simulink library "allblocks_alteradspbuilder2"  (Simulink 7.6)
(part 2 of 4)

  GND : S-Function  LoadFcn=alt_dspbuilder_load_block(gcb, 'BlockFactory', 'com.altera.dspbuilder.blockset.iobus.GND');  FunctionName=sGeneric  Parameters=SpecifyClock  EnableBusSupport=off  mask(GND AlteraBlockset){SpecifyClock=off, clock=}
      mask prompts: SpecifyClock "Specify Clock"
      mask help: A single bit which outputs a constant 0 value.
      mask init:
      | alt_dspbuilder_init('BlockFactory', 'com.altera.dspbuilder.blockset.iobus.GND', { get_param(gcb, 'SpecifyClock') clock });
      settings: CopyFcn=alt_dspbuilder_add_block(gcb, 'BlockFactory', 'com.altera.dspbuilder.blockset.iobus.GND');  DeleteFcn=com.altera.dspbuilder.simulation.Mask.delete(gcb);  UndoDeleteFcn=alt_dspbuilder_add_block(gcb, 'BlockFactory', 'com.altera.dspbuilder.blockset.iobus.GND');  PostSaveFcn=alt_dspbuilder_block_saved(gcb);  NameChangeFcn=alt_dspbuilder_block_renamed(gcb);
      mask Help: helpview(char(com.altera.dspbuilder.simulation.Cache.getBlockTemplate('BlockFactory', 'com.altera.dspbuilder.blockset.iobus.GND').getHelpFile))
      mask CallbackString: alt_dspbuilder_update_gui('BlockFactory', 'com.altera.dspbuilder.blockset.iobus.GND', 'SpecifyClock', 0);|
      mask Display:
      | plot([1 0 0 1], [1 1 0 0])
      | disp('0');
  Gain : S-Function  LoadFcn=alt_dspbuilder_load_block(gcb, 'BlockFactory', 'com.altera.dspbuilder.blockset.arithmetic.Gain');  FunctionName=sGeneric  Parameters=vgain BusType bwl bwr pipeline pipeline_display allowFloatingPointOverride logOutputs logFile MaskValue use_ena use_aclr lpm  EnableBusSupport=off  mask(Gain AlteraBlockset){vgain=2, BusType=Signed Integer, bwl=8, bwr=0, pipeline=1, pipeline_display=1, allowFloatingPointOverride=on, logOutputs=off, logFile=D:\\allblocks%5Falteradspbuilder2_Gain.fixedpointlog, MaskValue=1, use_ena=off, use_aclr=off, lpm=off}
      mask prompts: vgain "Gain Value"; BusType "Map Gain Value to Bus Type"; bwl "[Gain Value Number Of Bits].[]"; bwr "[].[Gain Value Number Of Bits]"; pipeline "Number Of Pipeline Stages"; pipeline_display "Number Of Pipeline Stages (Calculated)"; allowFloatingPointOverride "Allow Floating Point Override For This Block"; MaskValue "Clock Phase Selection"; use_ena "Use Enable Port (ena)"; use_aclr "Use Asynchronous Clear Port (aclr)"; lpm "Use LPM"
      mask help: Multiplies an input by a specified scalar gain factor.
      mask init:
      | alt_dspbuilder_init('BlockFactory', 'com.altera.dspbuilder.blockset.arithmetic.Gain', { vgain get_param(gcb, 'BusType') bwl bwr pipeline pipeline_display allowFloatingPointOverride logOutputs logFile MaskValue use_ena use_aclr lpm });
      settings: CopyFcn=alt_dspbuilder_add_block(gcb, 'BlockFactory', 'com.altera.dspbuilder.blockset.arithmetic.Gain');  DeleteFcn=com.altera.dspbuilder.simulation.Mask.delete(gcb);  UndoDeleteFcn=alt_dspbuilder_add_block(gcb, 'BlockFactory', 'com.altera.dspbuilder.blockset.arithmetic.Gain');  PostSaveFcn=alt_dspbuilder_block_saved(gcb);  NameChangeFcn=alt_dspbuilder_block_renamed(gcb);
      mask Help: helpview(char(com.altera.dspbuilder.simulation.Cache.getBlockTemplate('BlockFactory', 'com.altera.dspbuilder.blockset.arithmetic.Gain').getHelpFile))
      mask StyleString: edit,popup(Signed Integer|Unsigned Integer|Signed Fractional|Unsigned Fractional),edit,edit,edit,edit,checkbox,checkbox,edit,edit,checkbox,checkbox,checkbox
      mask CallbackString: |alt_dspbuilder_update_gui('BlockFactory', 'com.altera.dspbuilder.blockset.arithmetic.Gain', 'BusType', 1);|||||||||||
      mask TabNameString: Main,Main,Main,Main,Main,Main,Main,Main,Main,Optional Ports and Settings,Optional Ports and Settings,Optional Ports and Settings,Optional Ports and Settings
      mask Display:
      | port_label('input', 1, 'd');
      | port_label('output', 1, 'r');
      | plot([0 0 0 1 0], [0 1 0 0.5 1])
      | disp(2);
  Global Reset : S-Function  LoadFcn=alt_dspbuilder_load_block(gcb, 'BlockFactory', 'com.altera.dspbuilder.blockset.iobus.GlobalReset');  FunctionName=sGeneric  Parameters=SpecifyClock  EnableBusSupport=off  mask(GlobalReset AlteraBlockset){SpecifyClock=off, clock=}
      mask prompts: SpecifyClock "Specify Clock"
      mask help: Provides a single bit reset signal. All signals driven by the block are connected to the global reset for that clock domain. In simulation, this block outputs a constant 0.
      mask init:
      | alt_dspbuilder_init('BlockFactory', 'com.altera.dspbuilder.blockset.iobus.GlobalReset', { get_param(gcb, 'SpecifyClock') get_param(gcb, 'clock') });
      settings: CopyFcn=alt_dspbuilder_add_block(gcb, 'BlockFactory', 'com.altera.dspbuilder.blockset.iobus.GlobalReset');  DeleteFcn=com.altera.dspbuilder.simulation.Mask.delete(gcb);  UndoDeleteFcn=alt_dspbuilder_add_block(gcb, 'BlockFactory', 'com.altera.dspbuilder.blockset.iobus.GlobalReset');  PostSaveFcn=alt_dspbuilder_block_saved(gcb);  NameChangeFcn=alt_dspbuilder_block_renamed(gcb);
      mask Help: helpview(char(com.altera.dspbuilder.simulation.Cache.getBlockTemplate('BlockFactory', 'com.altera.dspbuilder.blockset.iobus.GlobalReset').getHelpFile))
      mask CallbackString: alt_dspbuilder_update_gui('BlockFactory', 'com.altera.dspbuilder.blockset.iobus.GlobalReset', 'SpecifyClock', 0);|alt_dspbuilder_update_gui('BlockFactory', 'com.altera.dspbuilder.blockset.iobus.GlobalReset', 'clock', 1);
      mask Display:
      | plot([1 0 0 1], [1 1 0 0])
      | disp('SCLR');
  HDL Entity : S-Function  LoadFcn=alt_dspbuilder_load_block(gcb, 'BlockFactory', 'com.altera.dspbuilder.blockset.altlab.HDLEntity');  FunctionName=sNoOp  Parameters=HDLFile clockname resetname useSubsystemPortName  EnableBusSupport=off  mask(HDL Entity AlteraBlockset){HDLFile=, clockname=, resetname=, useSubsystemPortName=off}
      mask prompts: HDLFile "HDL File Name"; clockname "Clock Name"; resetname "Reset Name"; useSubsystemPortName "HDL takes port names from Subsystem Inport/Outports"
      mask help:
      | This block is added to a black box simulation subsystem to specify the name of the HDL file that is substituted for the subsystem and
      | the names of the clock and reset ports for the subsystem. A HDL Entity block is usually automatically created by the Subsystem Builder Block.
      mask init:
      | alt_dspbuilder_init('BlockFactory', 'com.altera.dspbuilder.blockset.altlab.HDLEntity', { HDLFile clockname resetname useSubsystemPortName });
      settings: CopyFcn=alt_dspbuilder_add_block(gcb, 'BlockFactory', 'com.altera.dspbuilder.blockset.altlab.HDLEntity');  DeleteFcn=com.altera.dspbuilder.simulation.Mask.delete(gcb);  UndoDeleteFcn=alt_dspbuilder_add_block(gcb, 'BlockFactory', 'com.altera.dspbuilder.blockset.altlab.HDLEntity');  PostSaveFcn=alt_dspbuilder_block_saved(gcb);  NameChangeFcn=alt_dspbuilder_block_renamed(gcb);
      mask Help: helpview(char(com.altera.dspbuilder.simulation.Cache.getBlockTemplate('BlockFactory', 'com.altera.dspbuilder.blockset.altlab.HDLEntity').getHelpFile))
      mask Display: disp('');
  HDL Input : S-Function  LoadFcn=alt_dspbuilder_load_block(gcb, 'BlockFactory', 'com.altera.dspbuilder.blockset.altlab.HDLInput');  FunctionName=sInOut  Parameters=BusType bwl bwr externalType  EnableBusSupport=off  mask(HDL Input AlteraBlockset){BusType=Signed Integer, bwl=8, bwr=0, externalType=Inferred}
      mask prompts: BusType "Bus Type"; bwl "[number of bits].[]"; bwr "[].[number of bits]"; externalType "External Type"
      mask help:
      | This block should be connected directly to an output node in a subsystem. It is intended to be used with the Subsystem Builder and HDL Entity blocks for black box simulation.
      |
      | The type and bit width must match the type and bit width on the corresponding input port in the HDL file specified in the HDL Entity block. HDL Input blocks are automatically created by the Subsystem Builder block.
      mask init:
      | alt_dspbuilder_init('BlockFactory', 'com.altera.dspbuilder.blockset.altlab.HDLInput', { get_param(gcb, 'BusType') bwl bwr externalType });
      settings: CopyFcn=alt_dspbuilder_add_block(gcb, 'BlockFactory', 'com.altera.dspbuilder.blockset.altlab.HDLInput');  DeleteFcn=com.altera.dspbuilder.simulation.Mask.delete(gcb);  UndoDeleteFcn=alt_dspbuilder_add_block(gcb, 'BlockFactory', 'com.altera.dspbuilder.blockset.altlab.HDLInput');  PostSaveFcn=alt_dspbuilder_block_saved(gcb);  NameChangeFcn=alt_dspbuilder_block_renamed(gcb);
      mask Help: helpview(char(com.altera.dspbuilder.simulation.Cache.getBlockTemplate('BlockFactory', 'com.altera.dspbuilder.blockset.altlab.HDLInput').getHelpFile))
      mask StyleString: popup(Signed Integer|Unsigned Integer|Signed Fractional|Unsigned Fractional|Single Bit),edit,edit,popup(Inferred|Simulink Fixed Point Type|Double)
      mask CallbackString: alt_dspbuilder_update_gui('BlockFactory', 'com.altera.dspbuilder.blockset.altlab.HDLInput', 'BusType', 0);|||
      mask Display:
      | plot([0.17 0 0.83 1 0.83 0 0.17], [0.5 0 0 0.5 1 1 0.5])
      | plot([0.07 0.23 0.07 0.77 0.93  0.77], [0 0.5 1 1 0.5 0])
      | disp('i7:0')
  HDL Output : S-Function  LoadFcn=alt_dspbuilder_load_block(gcb, 'BlockFactory', 'com.altera.dspbuilder.blockset.altlab.HDLOutput');  FunctionName=sInOut  Parameters=BusType bwl bwr externalType  EnableBusSupport=off  mask(HDL Output AlteraBlockset){BusType=Signed Integer, bwl=8, bwr=0, externalType=Inferred}
      mask prompts: BusType "Bus Type"; bwl "[number of bits].[]"; bwr "[].[number of bits]"; externalType "External Type"
      mask help:
      | This block should be connected directly to an input node in a subsystem. It is intended to be used with the Subsystem Builder and HDL Entity blocks for black box simulation.
      |
      | The type and bit width must match the type and bit width on the corresponding output port in the HDL file specified in the HDL Entity block. HDL Output blocks are automatically created by the Subsystem Builder block.
      mask init:
      | alt_dspbuilder_init('BlockFactory', 'com.altera.dspbuilder.blockset.altlab.HDLOutput', { get_param(gcb, 'BusType') bwl bwr externalType });
      settings: CopyFcn=alt_dspbuilder_add_block(gcb, 'BlockFactory', 'com.altera.dspbuilder.blockset.altlab.HDLOutput');  DeleteFcn=com.altera.dspbuilder.simulation.Mask.delete(gcb);  UndoDeleteFcn=alt_dspbuilder_add_block(gcb, 'BlockFactory', 'com.altera.dspbuilder.blockset.altlab.HDLOutput');  PostSaveFcn=alt_dspbuilder_block_saved(gcb);  NameChangeFcn=alt_dspbuilder_block_renamed(gcb);
      mask Help: helpview(char(com.altera.dspbuilder.simulation.Cache.getBlockTemplate('BlockFactory', 'com.altera.dspbuilder.blockset.altlab.HDLOutput').getHelpFile))
      mask StyleString: popup(Signed Integer|Unsigned Integer|Signed Fractional|Unsigned Fractional|Single Bit),edit,edit,popup(Inferred|Simulink Fixed Point Type|Double)
      mask CallbackString: alt_dspbuilder_update_gui('BlockFactory', 'com.altera.dspbuilder.blockset.altlab.HDLOutput', 'BusType', 0);|||
      mask Display:
      | plot([0 0.17 1 0.83 1 0.17 0], [0.5 0 0 0.5 1 1 0.5])
      | plot([0.23 0.07 0.23 0.93 0.77 0.93], [0 0.5 1 1 0.5 0])
      | disp('o7:0')
  HDLImport : S-Function  LoadFcn=alt_dspbuilder_load_block(gcb, 'BlockFactory', 'com.altera.dspbuilder.blockset.altlab.HDLImport');  InitFcn=alt_dspbuilder_internal_init_blackbox_flow;  FunctionName=sGeneric  Parameters=entityName inNames inBwls inBwrs inTypes inDelayed outNames outBwls outBwrs outTypes resetNames resetTypes resetLengths xmlmapfile vofile src_file qpf_file TopLevelName UseQPF n_input_port n_output_port array_clocks use_systemC_model is_megacore use_dynamic_feedthrough_data use_alphabetical_port_ordering allowFloatingPointOverride  EnableBusSupport=off  mask(HDLImport AlteraBlockset){entityName=, inNames=, inBwls=, inBwrs=, inTypes=, inDelayed=, outNames=, outBwls=, outBwrs=, outTypes=, resetNames=, resetTypes=, resetLengths=, xmlmapfile=SimgenCMap.xml, vofile=test_core.vo, src_file=, qpf_file=, TopLevelName=, UseQPF=false, n_input_port=0, n_output_port=0, array_clocks=, use_systemC_model=off, is_megacore=off, use_dynamic_feedthrough_data=off, use_alphabetical_port_ordering=, allowFloatingPointOverride=off}
      mask prompts: entityName "Entity Name"; inNames "Input port names"; inBwls "Input Bitwidth lefts"; inBwrs "Input Bitwidth rights"; inTypes "Input Types"; inDelayed "Input Delayed Flags"; outNames "Output port names"; outBwls "Output Bitwidth lefts"; outBwrs "Output Bitwidth rights"; outTypes "Output Types"; resetNames "array_clocks"; resetTypes "array_clocks"; resetLengths "array_clocks"; use_systemC_model "Use SystemC bit-accurate model"
      mask help: Used to import supported VHDL or Verilog HDL components into DSP Builder, generating hardware and simulation models as required. You can either specify the HDL files directly, or select a Quartus II project file (.qpf) that defines the required HDL files. The HDL Import dialog box must be closed before simulation can start.
      mask init:
      | alt_dspbuilder_init('BlockFactory', 'com.altera.dspbuilder.blockset.altlab.HDLImport', { entityName inNames inBwls inBwrs inTypes inDelayed outNames outBwls outBwrs outTypes resetNames resetTypes resetLengths xmlmapfile vofile src_file qpf_file TopLevelName UseQPF n_input_port n_output_port array_clocks use_systemC_model is_megacore use_dynamic_feedthrough_data use_alphabetical_port_ordering allowFloatingPointOverride });
      settings: CopyFcn=alt_dspbuilder_add_block(gcb, 'BlockFactory', 'com.altera.dspbuilder.blockset.altlab.HDLImport');  DeleteFcn=com.altera.dspbuilder.simulation.Mask.delete(gcb);  UndoDeleteFcn=alt_dspbuilder_add_block(gcb, 'BlockFactory', 'com.altera.dspbuilder.blockset.altlab.HDLImport');  PostSaveFcn=alt_dspbuilder_block_saved(gcb);  NameChangeFcn=alt_dspbuilder_block_renamed(gcb);
      settings: OpenFcn=|
      | com.altera.dspbuilder.simulation.Mask.simpleInit('BlockFactory', 'com.altera.dspbuilder.blockset.altlab.HDLImport', bdroot(gcb), gcb);
      | alt_dspbuilder_internal_HDLimportlaunch(gcb, 0)
      mask Help: helpview(char(com.altera.dspbuilder.simulation.Cache.getBlockTemplate('BlockFactory', 'com.altera.dspbuilder.blockset.altlab.HDLImport').getHelpFile))
      mask Display: disp('HDL')
  HIL : S-Function  LoadFcn=alt_dspbuilder_load_block(gcb, 'BlockFactory', 'com.altera.dspbuilder.blockset.altlab.HardwareInTheLoop');  FunctionName=sGeneric  Parameters=entityName inNames inBwls inBwrs inTypes inDelayed outNames outBwls outBwrs outTypes resetNames resetTypes resetLengths InputCount InputNames InputWidth InputRepresentation InputExport InputFPP OutputCount OutputNames OutputWidth OutputRepresentation OutputExport OutputFPP JtagCable JtagDevice BurstMode BurstLength FrameMode SOP OutValid QuartusProject HilNewConfig ClockPinLocation ClockPinSource HilDeviceOnBoard DR_length dspbuilder_reset SLD_NODE_INFO AssertSclrBeforeSimulation SampleTime dspb_ver ResetLevel JtagCableName JtagDeviceName ResetNames ClockNames  EnableBusSupport=off  mask(HardwareInTheLoop AlteraBlockset){entityName=, inNames=, inBwls=, inBwrs=, inTypes=, inDelayed=, outNames=, outBwls=, outBwrs=, outTypes=, resetNames=, resetTypes=, resetLengths=, InputCount=0, InputNames=, InputWidth=0, InputRepresentation=b, InputExport=0, InputFPP=0, OutputCount=0, OutputNames=, OutputWidth=0, OutputRepresentation=0, OutputExport=0, OutputFPP=0, JtagCable=1, JtagDevice=1, BurstMode=off, BurstLength=0, FrameMode=off, SOP=0, OutValid=0, QuartusProject=0, HilNewConfig=0, ClockPinLocation=0, ClockPinSource=0, HilDeviceOnBoard=0, DR_length=0, dspbuilder_reset=1, SLD_NODE_INFO=0, AssertSclrBeforeSimulation=0, SampleTime=0, dspb_ver=0, ResetLevel=Active_High, JtagCableName=a, JtagDeviceName=b, ResetNames=, ClockNames=}
      mask prompts: entityName "Entity Name"; inNames "Input port names"; inBwls "Input Bitwidth lefts"; inBwrs "Input Bitwidth rights"; inTypes "Input Types"; inDelayed "Input Delayed Flags"; outNames "Output port names"; outBwls "Output Bitwidth lefts"; outBwrs "Output Bitwidth rights"; outTypes "Output Types"; resetNames "array_clocks"; resetTypes "array_clocks"; resetLengths "array_clocks"; InputCount "Input Count"; InputNames "Input Names"; InputWidth "Input Width"; InputRepresentation "Input Representation"; InputExport "Input Export"; InputFPP "Input FPP"; OutputCount "Output Count"; OutputNames "Output Names"; OutputWidth "Output Width"; OutputRepresentation "Output Representation"; OutputExport "Output Export"; OutputFPP "Output FPP"; JtagCable "JTAG Cable"; JtagDevice "JTAG Device"; BurstMode "Burst Mode"; BurstLength "Burst Length"; FrameMode "Frame Mode"; OutValid "Out Valid"; QuartusProject "Quartus Project"; HilNewConfig "HIL New Config"; ClockPinLocation "Clock Pin Location"; ClockPinSource "Clock Pin Source"; HilDeviceOnBoard "Hil Device On Board"; DR_length "DR Length"; dspbuilder_reset "DSP Builder Reset"; SLD_NODE_INFO "SLD NODE INFO"; AssertSclrBeforeSimulation "Assert Sclr Before Simulation"; SampleTime "Sample Time"; dspb_ver "DSP Builder Version"; ResetLevel "Reset Level"; JtagCableName "JTAG Cable Name"; JtagDeviceName "JTAG Device Name"; ResetNames "Reset Names"; ClockNames "Clock Names"
      mask help: The HIL (Hardware In the Loop) block allows you to use an FPGA as a simulation device inside a Simulink design. This configuration improves the simulation time, and also allows access to real hardware within a simulation.
      mask init:
      | alt_dspbuilder_init_hil('BlockFactory', 'com.altera.dspbuilder.blockset.altlab.HardwareInTheLoop', { entityName inNames inBwls inBwrs inTypes inDelayed outNames outBwls outBwrs outTypes resetNames resetTypes resetLengths InputCount InputNames InputWidth InputRepresentation InputExport InputFPP OutputCount OutputNames OutputWidth OutputRepresentation OutputExport OutputFPP JtagCable JtagDevice BurstMode BurstLength FrameMode SOP OutValid QuartusProject HilNewConfig ClockPinLocation ClockPinSource HilDeviceOnBoard DR_length dspbuilder_reset SLD_NODE_INFO AssertSclrBeforeSimulation SampleTime dspb_ver ResetLevel JtagCableName JtagDeviceName ResetNames ClockNames });
      settings: CopyFcn=alt_dspbuilder_add_block(gcb, 'BlockFactory', 'com.altera.dspbuilder.blockset.altlab.HardwareInTheLoop');  DeleteFcn=com.altera.dspbuilder.simulation.Mask.delete(gcb);  UndoDeleteFcn=alt_dspbuilder_add_block(gcb, 'BlockFactory', 'com.altera.dspbuilder.blockset.altlab.HardwareInTheLoop');  PostSaveFcn=alt_dspbuilder_block_saved(gcb);  NameChangeFcn=alt_dspbuilder_block_renamed(gcb);
      settings: OpenFcn=|
      | com.altera.dspbuilder.simulation.Mask.simpleInit('BlockFactory', 'com.altera.dspbuilder.blockset.altlab.HardwareInTheLoop', bdroot(gcb), gcb);
      | alt_dspbuilder_HilConfig('BLOCKNAME', gcb)
      mask Help: helpview(char(com.altera.dspbuilder.simulation.Cache.getBlockTemplate('BlockFactory', 'com.altera.dspbuilder.blockset.altlab.HardwareInTheLoop').getHelpFile))
      mask Display:
      | plot([-20],[0]);
      | plot([23],[26]);
      | plot([0 4 3 5 3 1 2 0],[0 3 3 6 6 3 3 0]);
      | plot([0 4 3 5 3 1 2 0],[20 23 23 26 26 23 23 20]);
      | disp(entityName);
  If Statement : S-Function  LoadFcn=alt_dspbuilder_load_block(gcb, 'BlockFactory', 'com.altera.dspbuilder.blockset.gatecontrol.IfStatement');  FunctionName=sGeneric  Parameters=user_inputs if_expression BusType bwl bwr pipeline_display use_else_output use_elseif_input  EnableBusSupport=off  mask(If Statement AlteraBlockset){user_inputs=4, if_expression=(a=b)|(c=d), BusType=Inferred, bwl=8, bwr=0, pipeline_display=1, use_else_output=off, use_elseif_input=off}
      mask prompts: user_inputs "Number Of Inputs"; if_expression "If Expression"; BusType "Data Bus Type"; bwl "[Number Of Bits].[]"; bwr "[].[Number Of Bits]"; pipeline_display "Number Of Pipeline Stages (Calculated)"; use_else_output "Use ELSE Output Port (false)"; use_elseif_input "Use ELSE IF Input Port (else)"
      mask help:
      | Outputs a '0' or '1' on port 'true' dependent on the evaluation of the given expression. (The output is '1' when the expression evaluates to true).
      |
      | The following operators can be used to build the expression:
      |
      | 	& 	AND
      | 	| 	OR
      | 	$ 	XOR
      | 	= 	Equal to
      | 	~ 	Not equal to
      | 	> 	Greater than
      | 	< 	Less than
      | 	()	Parentheses
      |
      | The following single-digit numerals can also be used:
      |
      |     0   zero
      |     1   one
      |
      | ELSE Output option: Create an output (false), based on an ELSE condition. (This will be '1' when the expression evaluates to false).
      | ELSE IF Input option: Create an input (else), which is a single bit used to cascade If Statement blocks to build IF {}, ELSE IF {} structures. This acts as an enable for the block.
      |
      | Note that the inputs (10 maximum) are annotated a,...,j and have the same (specified) type. The chosen type must be capable of expressing 0 and 1 exactly.
      mask init:
      | alt_dspbuilder_init('BlockFactory', 'com.altera.dspbuilder.blockset.gatecontrol.IfStatement', { user_inputs if_expression get_param(gcb, 'BusType') bwl bwr pipeline_display use_else_output use_elseif_input });
      settings: CopyFcn=alt_dspbuilder_add_block(gcb, 'BlockFactory', 'com.altera.dspbuilder.blockset.gatecontrol.IfStatement');  DeleteFcn=com.altera.dspbuilder.simulation.Mask.delete(gcb);  UndoDeleteFcn=alt_dspbuilder_add_block(gcb, 'BlockFactory', 'com.altera.dspbuilder.blockset.gatecontrol.IfStatement');  PostSaveFcn=alt_dspbuilder_block_saved(gcb);  NameChangeFcn=alt_dspbuilder_block_renamed(gcb);
      mask Help: helpview(char(com.altera.dspbuilder.simulation.Cache.getBlockTemplate('BlockFactory', 'com.altera.dspbuilder.blockset.gatecontrol.IfStatement').getHelpFile))
      mask StyleString: edit,edit,popup(Inferred|Signed Integer|Unsigned Integer|Signed Fractional|Unsigned Fractional|Single Bit),edit,edit,edit,checkbox,checkbox
      mask CallbackString: ||alt_dspbuilder_update_gui('BlockFactory', 'com.altera.dspbuilder.blockset.gatecontrol.IfStatement', 'BusType', 2);|||||
      mask TabNameString: Main,Main,Main,Main,Main,Main,Optional Ports,Optional Ports
      mask Display:
      | port_label('input', 1, 'a');
      | port_label('input', 2, 'b');
      | port_label('input', 3, 'c');
      | port_label('input', 4, 'd');
      | port_label('output', 1, 'true');
      | disp('IF (a=b)|(c=d)')
  Increment Decrement : S-Function  LoadFcn=alt_dspbuilder_load_block(gcb, 'BlockFactory', 'com.altera.dspbuilder.blockset.arithmetic.IncrementDecrement');  FunctionName=sGeneric  Parameters=BusType bwl bwr SpecifyClock clr_value direction phase_selection use_ena use_sclr pipeline_display  EnableBusSupport=off  mask(Increment Decrement AlteraBlockset){BusType=Signed Integer, bwl=8, bwr=8, SpecifyClock=off, clock=, clr_value=0, direction=Increment, phase_selection=1, use_ena=off, use_sclr=off, pipeline_display=1}
      mask prompts: BusType "Bus Type"; bwl "[Number Of Bits].[]"; bwr "[].[Number Of Bits]"; SpecifyClock "Specify Clock"; clr_value "Starting Value"; phase_selection "Clock Phase Selection"; use_ena "Use Enable Port (ena)"; use_sclr "Use Synchronous Clear Port (sclr)"; pipeline_display "Number Of Pipeline Stages (Calculated)"
      mask help:
      | Increments or decrements a value in time. The bus type and number of bits determines the type and size of the output from the block.
      | The output value increments or decrements by the smallest representable value; for integer types, the value always changes by 1.
      |
      | Direction specifies whether the value is incremented or decremented.
      | Starting Value specifies the initial output value of the block after a reset.
      | Clock Phase Selection is a binary string which sets the phases in which the block is enabled. For example:
      | 	0100	The delay block is enabled only on the 2nd phase of 4.
      mask init:
      | alt_dspbuilder_init('BlockFactory', 'com.altera.dspbuilder.blockset.arithmetic.IncrementDecrement', { get_param(gcb, 'BusType') bwl bwr get_param(gcb, 'SpecifyClock') clock clr_value direction phase_selection use_ena use_sclr pipeline_display });
      settings: CopyFcn=alt_dspbuilder_add_block(gcb, 'BlockFactory', 'com.altera.dspbuilder.blockset.arithmetic.IncrementDecrement');  DeleteFcn=com.altera.dspbuilder.simulation.Mask.delete(gcb);  UndoDeleteFcn=alt_dspbuilder_add_block(gcb, 'BlockFactory', 'com.altera.dspbuilder.blockset.arithmetic.IncrementDecrement');  PostSaveFcn=alt_dspbuilder_block_saved(gcb);  NameChangeFcn=alt_dspbuilder_block_renamed(gcb);
      mask Help: helpview(char(com.altera.dspbuilder.simulation.Cache.getBlockTemplate('BlockFactory', 'com.altera.dspbuilder.blockset.arithmetic.IncrementDecrement').getHelpFile))
      mask StyleString: popup(Signed Integer|Unsigned Integer|Signed Fractional|Unsigned Fractional),edit,edit,checkbox,edit,edit,popup(Increment|Decrement),edit,checkbox,checkbox,edit
      mask CallbackString: alt_dspbuilder_update_gui('BlockFactory', 'com.altera.dspbuilder.blockset.arithmetic.IncrementDecrement', 'BusType', 0);|||alt_dspbuilder_update_gui('BlockFactory', 'com.altera.dspbuilder.blockset.arithmetic.IncrementDecrement', 'SpecifyClock', 3);|||||||
      mask TabNameString: Main,Main,Main,Main,Main,Optional Ports and Settings,Optional Ports and Settings,Optional Ports and Settings,Optional Ports and Settings,Optional Ports and Settings,Optional Ports and Settings
      mask Display:
      | port_label('output', 1, 'c(7:0)');
      | plot([0 0.14 0.14 0.29 0.29 0.43 0.43 0.57 0.57 0.71 0.71 0.86 0.86 1], [0 0 0.17 0.17 0.33 0.33 0.5 0.5 1 1 1 1 1 1]);
  Input : S-Function  LoadFcn=alt_dspbuilder_load_block(gcb, 'BlockFactory', 'com.altera.dspbuilder.blockset.iobus.Input');  FunctionName=sInOut  Parameters=iofile BusType bwl bwr SpecifyClock externalType allowFloatingPointOverride logOutputs  EnableBusSupport=off  mask(Input AlteraBlockset){iofile=d:\\SJ\\nightly\\13.1\\162\\w32\\acds\\quartus\\dsp_builder\\bin\\mdllibrary\\tb_allblocks_alteradspbuilder2\\allblocks%5Falteradspbuilder2_Input.salt, BusType=Signed Integer, bwl=8, bwr=0, SpecifyClock=off, clock=, PORTTYPE=Input, externalType=Inferred, allowFloatingPointOverride=on, logOutputs=off}
      mask prompts: BusType "Bus Type"; bwl "[Number Of Bits].[]"; bwr "[].[Number Of Bits]"; SpecifyClock "Specify Clock"; PORTTYPE "TYPE"; externalType "External Type"; allowFloatingPointOverride "Allow Floating Point Override For This Block"
      mask help:
      | Defines the input boundary of a hardware system and casts floating-point Simulink signals (from generic Simulink blocks) to signed binary fractional format (feeding DSP Builder blocks).
      |
      | Choose from signed integer, unsigned integer or signed fractional representation.  The Simulink value is truncated to the nearest possible representation.
      mask init:
      | alt_dspbuilder_init_io('BlockFactory', 'com.altera.dspbuilder.blockset.iobus.Input', { iofile get_param(gcb, 'BusType') bwl bwr get_param(gcb, 'SpecifyClock') clock PORTTYPE externalType allowFloatingPointOverride logOutputs });
      settings: CopyFcn=alt_dspbuilder_add_block(gcb, 'BlockFactory', 'com.altera.dspbuilder.blockset.iobus.Input');  DeleteFcn=com.altera.dspbuilder.simulation.Mask.delete(gcb);  UndoDeleteFcn=alt_dspbuilder_add_block(gcb, 'BlockFactory', 'com.altera.dspbuilder.blockset.iobus.Input');  PreSaveFcn=alt_dspbuilder_internal_presave_block(gcb);  PostSaveFcn=alt_dspbuilder_block_saved(gcb);  NameChangeFcn=alt_dspbuilder_block_renamed(gcb);
      mask Help: helpview(char(com.altera.dspbuilder.simulation.Cache.getBlockTemplate('BlockFactory', 'com.altera.dspbuilder.blockset.iobus.Input').getHelpFile))
      mask StyleString: edit,popup(Signed Integer|Unsigned Integer|Signed Fractional|Unsigned Fractional|Single Bit),edit,edit,checkbox,edit,edit,popup(Inferred|Simulink Fixed Point Type|Double),checkbox,checkbox
      mask CallbackString: |alt_dspbuilder_update_gui('BlockFactory', 'com.altera.dspbuilder.blockset.iobus.Input', 'BusType', 1);|||alt_dspbuilder_update_gui('BlockFactory', 'com.altera.dspbuilder.blockset.iobus.Input', 'SpecifyClock', 4);|||||
      mask Display:
      | plot([-25 15 25 15 -25 -25]*1, [0 0 -10 -20 -20 0] - 0);
      | plot([11 21 11]*1, [0 -10 -20] - 0);
      | text(0, -10, 'i7:0', 'horizontalAlignment','center','verticalAlignment','middle');
  Integrator : S-Function  LoadFcn=alt_dspbuilder_load_block(gcb, 'BlockFactory', 'com.altera.dspbuilder.blockset.arithmetic.Integrator');  FunctionName=sGeneric  Parameters=bwl depth pipeline_display use_ena use_sclr allowFloatingPointOverride logOutputs logFile  EnableBusSupport=off  mask(Integrator AlteraBlockset){bwl=20, depth=1, pipeline_display=1, use_ena=on, use_sclr=on, allowFloatingPointOverride=on, logOutputs=off, logFile=D:\\allblocks%5Falteradspbuilder2_Integrator.fixedpointlog}
      mask prompts: bwl "Number of Bits"; pipeline_display "Number Of Pipeline Stages (Calculated)"; use_ena "Use Enable Port (ena)"; use_sclr "Use Synchronous Clear Port (sclr)"; allowFloatingPointOverride "Allow Floating Point Override For This Block"
      mask help:
      | A signed integer integrator using the equation q(n+D) = q(n) + d(n)
      | where D is the delay parameter.
      mask init:
      | alt_dspbuilder_init('BlockFactory', 'com.altera.dspbuilder.blockset.arithmetic.Integrator', { bwl depth pipeline_display use_ena use_sclr allowFloatingPointOverride logOutputs logFile });
      settings: CopyFcn=alt_dspbuilder_add_block(gcb, 'BlockFactory', 'com.altera.dspbuilder.blockset.arithmetic.Integrator');  DeleteFcn=com.altera.dspbuilder.simulation.Mask.delete(gcb);  UndoDeleteFcn=alt_dspbuilder_add_block(gcb, 'BlockFactory', 'com.altera.dspbuilder.blockset.arithmetic.Integrator');  PostSaveFcn=alt_dspbuilder_block_saved(gcb);  NameChangeFcn=alt_dspbuilder_block_renamed(gcb);
      mask Help: helpview(char(com.altera.dspbuilder.simulation.Cache.getBlockTemplate('BlockFactory', 'com.altera.dspbuilder.blockset.arithmetic.Integrator').getHelpFile))
      mask TabNameString: Main,Main,Main,Optional Ports,Optional Ports,Optional Ports,Optional Ports,Optional Ports
      mask Display:
      | port_label('input', 1, 'd(19:0)');
      | port_label('input', 2, 'ena');
      | port_label('input', 3, 'sclr');
      | port_label('output', 1, 'q(19:0)');
      | dpoly([zeros(1,1) 1],[1 zeros(1,0) -1],'z-');
  LFSR Sequence : S-Function  LoadFcn=alt_dspbuilder_load_block(gcb, 'BlockFactory', 'com.altera.dspbuilder.blockset.gatecontrol.LFSRSequence');  FunctionName=sGeneric  Parameters=length feedback_structure feedback_gate_type initial_reg_val_hex initial_reg_val_bin poly_tap_seq poly_tap_seq_bin SpecifyClock use_parallel_out use_ena use_sclr  EnableBusSupport=off  mask(LFSR Sequence AlteraBlockset){length=10, feedback_structure=External n-inputs gate (many-to-one), feedback_gate_type=XOR, initial_reg_val_hex=FFFFFFFF, initial_reg_val_bin=1111111111, poly_tap_seq=[3 10], poly_tap_seq_bin=1000000100, SpecifyClock=off, clock=, use_parallel_out=off, use_ena=off, use_sclr=off}
      mask prompts: length "LFSR Length"; feedback_structure "Feedback Structure"; feedback_gate_type "Feedback Gate Type"; initial_reg_val_hex "Initial Register Value (Hex)"; poly_tap_seq "Primitive Polynomial Tap Sequence"; SpecifyClock "Specify Clock"; use_parallel_out "Use Parallel Output (pout)"; use_ena "Use Enable Port (ena)"; use_sclr "Use Synchronous Clear Port (sclr)"
      mask help:
      | The LFSR Sequence block implements a linear feedback shift register which shifts one bit across L registers. The register output bits are shifted in the direction of LSB to MSB, with the output sout connected to the MSB of the shift register. The register output bits can optionally be XORed or XNORed together.
      |
      | The LFSR is initialized to the Initial Register Value. If this value is larger than representable in the shift register (set by LFSR Length) the unrepresentable bits are truncated.
      |
      | The Primitive Polynomial Tap Sequence describes where the taps will be in the shift register, 1 denotes the LSB, and the LFSR Length value denotes the MSB. The LFSR block must have a minimum of 2 taps.
      mask init:
      | alt_dspbuilder_init('BlockFactory', 'com.altera.dspbuilder.blockset.gatecontrol.LFSRSequence', { length get_param(gcb, 'feedback_structure') get_param(gcb, 'feedback_gate_type') initial_reg_val_hex initial_reg_val_bin poly_tap_seq poly_tap_seq_bin get_param(gcb, 'SpecifyClock') clock use_parallel_out use_ena use_sclr });
      settings: CopyFcn=alt_dspbuilder_add_block(gcb, 'BlockFactory', 'com.altera.dspbuilder.blockset.gatecontrol.LFSRSequence');  DeleteFcn=com.altera.dspbuilder.simulation.Mask.delete(gcb);  UndoDeleteFcn=alt_dspbuilder_add_block(gcb, 'BlockFactory', 'com.altera.dspbuilder.blockset.gatecontrol.LFSRSequence');  PostSaveFcn=alt_dspbuilder_block_saved(gcb);  NameChangeFcn=alt_dspbuilder_block_renamed(gcb);
      mask Help: helpview(char(com.altera.dspbuilder.simulation.Cache.getBlockTemplate('BlockFactory', 'com.altera.dspbuilder.blockset.gatecontrol.LFSRSequence').getHelpFile))
      mask StyleString: edit,popup(External n-inputs gate (many-to-one)|Internal two-inputs gate (one-to-many)),popup(XOR|XNOR),edit,edit,edit,edit,checkbox,edit,checkbox,checkbox,checkbox
      mask CallbackString: |alt_dspbuilder_update_gui('BlockFactory', 'com.altera.dspbuilder.blockset.gatecontrol.LFSRSequence', 'feedback_structure', 1);|alt_dspbuilder_update_gui('BlockFactory', 'com.altera.dspbuilder.blockset.gatecontrol.LFSRSequence', 'feedback_gate_type', 2);|||||alt_dspbuilder_update_gui('BlockFactory', 'com.altera.dspbuilder.blockset.gatecontrol.LFSRSequence', 'SpecifyClock', 7);||||
      mask TabNameString: Main,Main,Main,Main,Main,Main,Main,Main,Main,Optional Ports,Optional Ports,Optional Ports
      mask Display:
      | port_label('output', 1, 'sout');
      | disp('x^{10}+x^{3}+1' ,'texmode','on');
  LUT : S-Function  LoadFcn=alt_dspbuilder_load_block(gcb, 'BlockFactory', 'com.altera.dspbuilder.blockset.storage.LUT');  FunctionName=sGeneric  Parameters=addr_width BusType bwl bwr init_array allowFloatingPointOverride logOutputs logFile use_ena reg_data use_lpm reg_addr ram_type pipeline_display  EnableBusSupport=off  mask(LUT AlteraBlockset){addr_width=3, BusType=Signed Integer, bwl=8, bwr=0, init_array=[0:1:7], allowFloatingPointOverride=on, logOutputs=off, logFile=D:\\allblocks%5Falteradspbuilder2_LUT.fixedpointlog, use_ena=off, reg_data=off, use_lpm=on, reg_addr=on, ram_type=AUTO, pipeline_display=1}
      mask prompts: addr_width "Address Width"; BusType "Data Type"; bwl "[Number Of Bits].[]"; bwr "[].[Number Of Bits]"; init_array "MATLAB array"; allowFloatingPointOverride "Allow Floating Point Override For This Block"; use_ena "Use Enable Port (ena) when data or address is registered"; reg_data "Register Data"; use_lpm "Use LPM"; reg_addr "Register Address"; ram_type "Memory Block Type"; pipeline_display "Number Of Pipeline Stages (Calculated)"
      mask help:
      | The LUT block stores data as 2^(address width) words of data in a look-up table. The values of the words are specified in the data vector field as a MATLAB array.
      |
      | The MATLAB Array parameter must be a one dimensional MATLAB array with a length smaller than 2^(address width). The array can be specified from the MATLAB workspace or directly in the MATLAB Array box.
      |
      | The input address bus must be unsigned.
      |
      | Note that for LPM the input address is always registered and not all memory options are available for all families.
      mask init:
      | alt_dspbuilder_init('BlockFactory', 'com.altera.dspbuilder.blockset.storage.LUT', { addr_width get_param(gcb, 'BusType') bwl bwr init_array allowFloatingPointOverride logOutputs logFile use_ena reg_data get_param(gcb, 'use_lpm') reg_addr ram_type pipeline_display });
      settings: CopyFcn=alt_dspbuilder_add_block(gcb, 'BlockFactory', 'com.altera.dspbuilder.blockset.storage.LUT');  DeleteFcn=com.altera.dspbuilder.simulation.Mask.delete(gcb);  UndoDeleteFcn=alt_dspbuilder_add_block(gcb, 'BlockFactory', 'com.altera.dspbuilder.blockset.storage.LUT');  PostSaveFcn=alt_dspbuilder_block_saved(gcb);  NameChangeFcn=alt_dspbuilder_block_renamed(gcb);
      mask Help: helpview(char(com.altera.dspbuilder.simulation.Cache.getBlockTemplate('BlockFactory', 'com.altera.dspbuilder.blockset.storage.LUT').getHelpFile))
      mask StyleString: edit,popup(Signed Integer|Unsigned Integer|Signed Fractional|Unsigned Fractional|Single Bit),edit,edit,edit,checkbox,checkbox,edit,checkbox,checkbox,checkbox,checkbox,popup(AUTO|M9K|M10K|M20K|MLAB|M144K),edit
      mask CallbackString: |alt_dspbuilder_update_gui('BlockFactory', 'com.altera.dspbuilder.blockset.storage.LUT', 'BusType', 1);|||||||||alt_dspbuilder_update_gui('BlockFactory', 'com.altera.dspbuilder.blockset.storage.LUT', 'use_lpm', 10);|||
      mask TabNameString: Main,Main,Main,Main,Main,Main,Main,Main,Implementation,Implementation,Implementation,Implementation,Implementation,Implementation
      mask Display:
      | port_label('input', 1, '(2:0)');
      | port_label('output', 1, 'q(7:0)');
      | plot([0 1 0.43 0.43 0.71 0.71 0.71 0.43 0.43 0.71 0.71 0.43 0.43 0.71 0.71 0.43 0.43 0.71 0.71 0.43], [0 0 0 1 1 0 0.125 0.125 0.25 0.25 0.375 0.375 0.5 0.5 0.625 0.625 0.75 0.75 0.875 0.875])
  Logical Bit Operator : S-Function  LoadFcn=alt_dspbuilder_load_block(gcb, 'BlockFactory', 'com.altera.dspbuilder.blockset.gatecontrol.LogicalBitOp');  FunctionName=sGeneric  Parameters=LogicalOperator user_inputs pipeline_display  EnableBusSupport=off  mask(Logical Bit Operator AlteraBlockset){LogicalOperator=AND, user_inputs=2, pipeline_display=0}
      mask prompts: LogicalOperator "Logical Operation"; user_inputs "Number Of Inputs"; pipeline_display "Number Of Pipeline Stages (Calculated)"
      mask help: Performs logical operations on single-bit inputs. You can specify a variable number of inputs. If the integer is positive, it is interpreted as a boolean 1, otherwise it is interpreted as 0. The number of inputs is variable.
      mask init:
      | alt_dspbuilder_init('BlockFactory', 'com.altera.dspbuilder.blockset.gatecontrol.LogicalBitOp', { get_param(gcb, 'LogicalOperator') user_inputs pipeline_display });
      settings: CopyFcn=alt_dspbuilder_add_block(gcb, 'BlockFactory', 'com.altera.dspbuilder.blockset.gatecontrol.LogicalBitOp');  DeleteFcn=com.altera.dspbuilder.simulation.Mask.delete(gcb);  UndoDeleteFcn=alt_dspbuilder_add_block(gcb, 'BlockFactory', 'com.altera.dspbuilder.blockset.gatecontrol.LogicalBitOp');  PostSaveFcn=alt_dspbuilder_block_saved(gcb);  NameChangeFcn=alt_dspbuilder_block_renamed(gcb);
      mask Help: helpview(char(com.altera.dspbuilder.simulation.Cache.getBlockTemplate('BlockFactory', 'com.altera.dspbuilder.blockset.gatecontrol.LogicalBitOp').getHelpFile))
      mask StyleString: popup(AND|OR|XOR|NAND|NOR|NOT),edit,edit
      mask CallbackString: alt_dspbuilder_update_gui('BlockFactory', 'com.altera.dspbuilder.blockset.gatecontrol.LogicalBitOp', 'LogicalOperator', 0);||
      mask Display:
      | plot([-exp((pi/2:.1:1.5*pi)*i) -1+i -1-i 0-i])
      | 
      | 
      | 
      | 
      | 
      | 
      | 
      | disp('AND')
  Logical Bus Operator : S-Function  LoadFcn=alt_dspbuilder_load_block(gcb, 'BlockFactory', 'com.altera.dspbuilder.blockset.gatecontrol.LogicalBusOp');  FunctionName=sGeneric  Parameters=BusType bwl bwr LogicalOp_text mask_value_num shift_amount force_sign_ext pipeline_display  EnableBusSupport=off  mask(Logical Bus Operator AlteraBlockset){BusType=Signed Fractional, bwl=8, bwr=0, LogicalOp_text=AND, mask_value_num=-5, shift_amount=3, force_sign_ext=on, pipeline_display=0}
      mask prompts: BusType "Bus Type"; bwl "[Number Of Bits].[]"; bwr "[].[Number Of Bits]"; LogicalOp_text "Logical Operation"; mask_value_num "Mask Value"; shift_amount "Number of Bits to Shift"; force_sign_ext "Sign Extend (if right shifting signed data)"; pipeline_display "Number Of Pipeline Stages (Calculated)"
      mask help:
      | Performs logical operations on a bus such as AND, OR, XOR, and invert. You can perform masking by entering a mask value in decimal notation, or a shift (or rotate) operation by entering a number of bits.
      |
      | Note that by default the right shifting operation preserves the input data sign (for signed inputs).
      mask init:
      | alt_dspbuilder_init('BlockFactory', 'com.altera.dspbuilder.blockset.gatecontrol.LogicalBusOp', { get_param(gcb, 'BusType') bwl bwr get_param(gcb, 'LogicalOp_text') mask_value_num shift_amount force_sign_ext pipeline_display });
      settings: CopyFcn=alt_dspbuilder_add_block(gcb, 'BlockFactory', 'com.altera.dspbuilder.blockset.gatecontrol.LogicalBusOp');  DeleteFcn=com.altera.dspbuilder.simulation.Mask.delete(gcb);  UndoDeleteFcn=alt_dspbuilder_add_block(gcb, 'BlockFactory', 'com.altera.dspbuilder.blockset.gatecontrol.LogicalBusOp');  PostSaveFcn=alt_dspbuilder_block_saved(gcb);  NameChangeFcn=alt_dspbuilder_block_renamed(gcb);
      mask Help: helpview(char(com.altera.dspbuilder.simulation.Cache.getBlockTemplate('BlockFactory', 'com.altera.dspbuilder.blockset.gatecontrol.LogicalBusOp').getHelpFile))
      mask StyleString: popup(Signed Integer|Unsigned Integer|Signed Fractional|Unsigned Fractional),edit,edit,popup(AND|OR|XOR|Invert|Shift Left|Shift Right|Rotate Left|Rotate Right),edit,edit,checkbox,edit
      mask CallbackString: alt_dspbuilder_update_gui('BlockFactory', 'com.altera.dspbuilder.blockset.gatecontrol.LogicalBusOp', 'BusType', 0);|||alt_dspbuilder_update_gui('BlockFactory', 'com.altera.dspbuilder.blockset.gatecontrol.LogicalBusOp', 'LogicalOp_text', 3);||||
      mask Display:
      | port_label('input', 1, 'd[8]:[0]');
      | port_label('output', 1, 'q[8]:[0]');
      | 
      | fprintf('AND\n11111011');
  Logical Reduce Operator : S-Function  LoadFcn=alt_dspbuilder_load_block(gcb, 'BlockFactory', 'com.altera.dspbuilder.blockset.gatecontrol.LogicalReduceOp');  FunctionName=sGeneric  Parameters=BusType bwl bwr LogicalOperator pipeline_display  EnableBusSupport=off  mask(Logical Reduce Operator AlteraBlockset){BusType=Signed Integer, bwl=8, bwr=0, LogicalOperator=AND, pipeline_display=0}
      mask prompts: BusType "Bus Type"; bwl "[Number Of Bits].[]"; bwr "[].[Number Of Bits]"; LogicalOperator "Logical Reduction Operation"; pipeline_display "Number Of Pipeline Stages (Calculated)"
      mask help: Performs logical reduction operations on a bus such as AND, OR and XOR. The logical operation is applied bit-wise to the input bus to give a single bit result.
      mask init:
      | alt_dspbuilder_init('BlockFactory', 'com.altera.dspbuilder.blockset.gatecontrol.LogicalReduceOp', { get_param(gcb, 'BusType') bwl bwr LogicalOperator pipeline_display });
      settings: CopyFcn=alt_dspbuilder_add_block(gcb, 'BlockFactory', 'com.altera.dspbuilder.blockset.gatecontrol.LogicalReduceOp');  DeleteFcn=com.altera.dspbuilder.simulation.Mask.delete(gcb);  UndoDeleteFcn=alt_dspbuilder_add_block(gcb, 'BlockFactory', 'com.altera.dspbuilder.blockset.gatecontrol.LogicalReduceOp');  PostSaveFcn=alt_dspbuilder_block_saved(gcb);  NameChangeFcn=alt_dspbuilder_block_renamed(gcb);
      mask Help: helpview(char(com.altera.dspbuilder.simulation.Cache.getBlockTemplate('BlockFactory', 'com.altera.dspbuilder.blockset.gatecontrol.LogicalReduceOp').getHelpFile))
      mask StyleString: popup(Inferred|Signed Integer|Unsigned Integer|Signed Fractional|Unsigned Fractional),edit,edit,popup(AND|OR|XOR|NAND|NOR),edit
      mask CallbackString: alt_dspbuilder_update_gui('BlockFactory', 'com.altera.dspbuilder.blockset.gatecontrol.LogicalReduceOp', 'BusType', 0);||||
      mask Display:
      | port_label('input', 1, 'd(7:0)');
      | port_label('output', 1, 'q');
      | fprintf('AND');
  Magnitude : S-Function  LoadFcn=alt_dspbuilder_load_block(gcb, 'BlockFactory', 'com.altera.dspbuilder.blockset.arithmetic.Magnitude');  FunctionName=sGeneric  Parameters=pipeline_display  EnableBusSupport=off  mask(Magnitude AlteraBlockset){pipeline_display=0}
      mask prompts: pipeline_display "Number Of Pipeline Stages (Calculated)"
      mask help: Returns the absolute value of the incoming signed binary fractional bus.
      mask init:
      | alt_dspbuilder_init('BlockFactory', 'com.altera.dspbuilder.blockset.arithmetic.Magnitude', { pipeline_display });
      settings: CopyFcn=alt_dspbuilder_add_block(gcb, 'BlockFactory', 'com.altera.dspbuilder.blockset.arithmetic.Magnitude');  DeleteFcn=com.altera.dspbuilder.simulation.Mask.delete(gcb);  UndoDeleteFcn=alt_dspbuilder_add_block(gcb, 'BlockFactory', 'com.altera.dspbuilder.blockset.arithmetic.Magnitude');  PostSaveFcn=alt_dspbuilder_block_saved(gcb);  NameChangeFcn=alt_dspbuilder_block_renamed(gcb);
      mask Help: helpview(char(com.altera.dspbuilder.simulation.Cache.getBlockTemplate('BlockFactory', 'com.altera.dspbuilder.blockset.arithmetic.Magnitude').getHelpFile))
      mask Display: disp('|a|');
  Memory Delay : S-Function  LoadFcn=alt_dspbuilder_load_block(gcb, 'BlockFactory', 'com.altera.dspbuilder.blockset.storage.MemDelay');  FunctionName=sGeneric  Parameters=BusType bwl bwr pipeline pipeline_display ram_type use_ena use_sclr allowFloatingPointOverride logOutputs logFile  EnableBusSupport=off  mask(Memory Delay AlteraBlockset){BusType=Inferred, bwl=8, bwr=0, pipeline=1, pipeline_display=1, ram_type=AUTO, use_ena=off, use_sclr=off, allowFloatingPointOverride=on, logOutputs=off, logFile=D:\\allblocks%5Falteradspbuilder2_Memory+Delay.fixedpointlog}
      mask prompts: BusType "Data Type"; bwl "[Number Of Bits].[]"; bwr "[].[Number Of Bits]"; pipeline "Number Of Pipeline Stages"; pipeline_display "Number Of Pipeline Stages (Calculated)"; ram_type "Memory Block Type"; use_ena "Use Enable Port (ena)"; use_sclr "Use Asynchronous Clear Port (aclr)"; allowFloatingPointOverride "Allow Floating Point Override For This Block"
      mask help:
      | Implements a shift register that uses the Altera device's embedded memory blocks, when possible. You should typically use this block for delays greater than 3.
      |
      | Note that not all memory options are available for all device families.
      mask init:
      | alt_dspbuilder_init('BlockFactory', 'com.altera.dspbuilder.blockset.storage.MemDelay', { get_param(gcb, 'BusType') bwl bwr pipeline pipeline_display ram_type use_ena use_sclr allowFloatingPointOverride logOutputs logFile });
      settings: CopyFcn=alt_dspbuilder_add_block(gcb, 'BlockFactory', 'com.altera.dspbuilder.blockset.storage.MemDelay');  DeleteFcn=com.altera.dspbuilder.simulation.Mask.delete(gcb);  UndoDeleteFcn=alt_dspbuilder_add_block(gcb, 'BlockFactory', 'com.altera.dspbuilder.blockset.storage.MemDelay');  PostSaveFcn=alt_dspbuilder_block_saved(gcb);  NameChangeFcn=alt_dspbuilder_block_renamed(gcb);
      mask Help: helpview(char(com.altera.dspbuilder.simulation.Cache.getBlockTemplate('BlockFactory', 'com.altera.dspbuilder.blockset.storage.MemDelay').getHelpFile))
      mask StyleString: popup(Inferred|Signed Integer|Unsigned Integer|Signed Fractional|Unsigned Fractional),edit,edit,edit,edit,popup(AUTO|M9K|M10K|M20K|MLAB|M144K),checkbox,checkbox,checkbox,checkbox,edit
      mask CallbackString: alt_dspbuilder_update_gui('BlockFactory', 'com.altera.dspbuilder.blockset.storage.MemDelay', 'BusType', 0);||||||||||
      mask TabNameString: Main,Main,Main,Main,Main,Main,Optional Ports,Optional Ports,Optional Ports,Optional Ports,Optional Ports
      mask Display:
      | port_label('input', 1, 'd');
      | port_label('output', 1, 'q');
      | disp('z^{-1}','texmode','on');
      | text(0.5,0.1,'AUTO');
  Multi-Rate DFF : S-Function  LoadFcn=alt_dspbuilder_load_block(gcb, 'BlockFactory', 'com.altera.dspbuilder.blockset.RateChange.MultiRateDff');  FunctionName=sMultiRate  Parameters=pipeline UseBaseClock clock use_ena use_sclr  EnableBusSupport=off  mask(Multi-Rate DFF AlteraBlockset){pipeline=1, UseBaseClock=on, clock=clock, use_ena=off, use_sclr=off}
      mask prompts: pipeline "Number of Pipeline Stages"; UseBaseClock "Use Base Clock"; clock "Clock Name"; use_ena "Use Enable Port (ena)"; use_sclr "Use Synchronous Clear Port (sclr)"
      mask help:
      | Implements a D-type flipflop that is typically used to specify sample rate transitions.
      |
      | A Clock block must be added to the top level design to specify the various sample times when you use the Multi-Rate DFF block.
      mask init:
      | alt_dspbuilder_init('BlockFactory', 'com.altera.dspbuilder.blockset.RateChange.MultiRateDff', { pipeline get_param(gcb, 'UseBaseClock') clock get_param(gcb, 'use_ena') get_param(gcb, 'use_sclr') });
      settings: CopyFcn=alt_dspbuilder_add_block(gcb, 'BlockFactory', 'com.altera.dspbuilder.blockset.RateChange.MultiRateDff');  DeleteFcn=com.altera.dspbuilder.simulation.Mask.delete(gcb);  UndoDeleteFcn=alt_dspbuilder_add_block(gcb, 'BlockFactory', 'com.altera.dspbuilder.blockset.RateChange.MultiRateDff');  PostSaveFcn=alt_dspbuilder_block_saved(gcb);  NameChangeFcn=alt_dspbuilder_block_renamed(gcb);
      mask Help: helpview(char(com.altera.dspbuilder.simulation.Cache.getBlockTemplate('BlockFactory', 'com.altera.dspbuilder.blockset.RateChange.MultiRateDff').getHelpFile))
      mask CallbackString: |alt_dspbuilder_update_gui('BlockFactory', 'com.altera.dspbuilder.blockset.RateChange.MultiRateDff', 'UseBaseClock', 1);||alt_dspbuilder_update_gui('BlockFactory', 'com.altera.dspbuilder.blockset.RateChange.MultiRateDff', 'use_ena', 3);|alt_dspbuilder_update_gui('BlockFactory', 'com.altera.dspbuilder.blockset.RateChange.MultiRateDff', 'use_sclr', 4);
      mask TabNameString: Main,Main,Main,Optional Ports,Optional Ports
      mask Display:
      | port_label('input', 1, 'd');
      | port_label('output', 1, 'q');
      | fprintf('DFF\n(20 ns)');
  Multiple Port External RAM : S-Function  InitFcn=alt_dspbuilder_update_external_RAM();  StartFcn=alt_dspbuilder_internal_externalRAMWarning  FunctionName=sExternalRAM  Parameters=WRITE_INTERFACES READ_INTERFACES DATA_WIDTH ADDRESS_WIDTH WAIT_STATES_PER_WRITE MAXIMUM_LATENCY SIZE OFFSET  EnableBusSupport=off  mask{WRITE_INTERFACES=1, READ_INTERFACES=1, DATA_WIDTH=32, ADDRESS_WIDTH=8, WAIT_STATES_PER_WRITE=0, MAXIMUM_LATENCY=1, SIZE=100, OFFSET=0}
      mask prompts: WRITE_INTERFACES "Number of Write Interfaces"; READ_INTERFACES "Number of Read Interfaces"; DATA_WIDTH "Data Width"; ADDRESS_WIDTH "Address Width"; WAIT_STATES_PER_WRITE "Wait States Per Write"; MAXIMUM_LATENCY "Maximum Latency"
      mask help:
      | This is a simulation model of an external RAM block.  It can be used to store and retrieve data from a range of addresses.  It is designed specifically to work with the DSP Builder Video and Image Processing blocks, but may be used for other purposes.
      |
      | As it is a simulation only block, it will not generate HDL when SignalCompiler is run.
      |
      | Parameters
      | =========
      | Data Width - the number of bits used for the data (8,16, 32, 64 or 128 bits only)
      | Address Width - number of bits used for the address (between 1 and 32)
      | Wait States Per Write - choose a fixed number of wait states for each write transfer (between 0 to 10)
      | Maximum Latency - set the latency for pipelined read transfer (between 1 and 255)
      | Size, Offset - to use a range of addresses, choose an offset (start address) and size (number of addresses).  The size added to the offset must be less than 2 ^ address width).
      |
      | Note : If 64 or 128 bits are selected for the data width, the block will attempt to register a Simulink fixed point type of the corresponding width.  This will only work if a valid fixed point license is present on the user's machine.  Please refer to the Simulink help for more information about fixed point licenses.
      mask Help: helpview(fullfile(alt_dspbuilder_get_quartus_rootdir, 'dsp_builder', 'docs', 'MultiplePortExternalRAM.html'))
      mask Display:
      | port_label('input', 1, 'WriteData1');
      | port_label('input', 2, 'WriteAddress1');
      | port_label('input', 3, 'WriteEnable1');
      | port_label('input', 4, 'WriteBurstCount1');
      | port_label('output', 1, 'WriteWaitRequest1');
      | port_label('input', 5, 'ReadAddress1');
      | port_label('input', 6, 'ReadEnable1');
      | port_label('input', 7, 'ReadBurstCount1');
      | port_label('output', 2, 'ReadData1');
      | port_label('output', 3, 'ReadDataValid1');
      | port_label('output', 4, 'ReadWaitRequest1');
  Multiplexer : S-Function  LoadFcn=alt_dspbuilder_load_block(gcb, 'BlockFactory', 'com.altera.dspbuilder.blockset.gatecontrol.Multiplexer');  FunctionName=sGeneric  Parameters=numInputs pipeline oneHot pipeline_display use_ena use_aclr allowFloatingPointOverride logOutputs logFile  EnableBusSupport=off  mask(Multiplexer AlteraBlockset){numInputs=6, pipeline=0, oneHot=off, pipeline_display=0, use_ena=off, use_aclr=off, allowFloatingPointOverride=on, logOutputs=off, logFile=D:\\allblocks%5Falteradspbuilder2_Multiplexer.fixedpointlog}
      mask prompts: numInputs "Number Of Input Data Lines"; pipeline "Number Of Pipeline Stages"; oneHot "One Hot Select Bus"; pipeline_display "Number Of Pipeline Stages (Calculated)"; use_ena "Use Enable Port (ena)"; use_aclr "Use Asynchronous Clear Port (aclr)"; allowFloatingPointOverride "Allow Floating Point Override For This Block"
      mask help:
      | Operates as either a one-hot or full binary bus multiplexer with one select control.
      |
      | The output width of the multiplexer is equal to the maximum of the widths of the input data lines. The block works on any data type and sign extends the inputs if there is a bit width mismatch.
      mask init:
      | alt_dspbuilder_init('BlockFactory', 'com.altera.dspbuilder.blockset.gatecontrol.Multiplexer', { numInputs pipeline oneHot pipeline_display use_ena use_aclr allowFloatingPointOverride logOutputs logFile });
      settings: CopyFcn=alt_dspbuilder_add_block(gcb, 'BlockFactory', 'com.altera.dspbuilder.blockset.gatecontrol.Multiplexer');  DeleteFcn=com.altera.dspbuilder.simulation.Mask.delete(gcb);  UndoDeleteFcn=alt_dspbuilder_add_block(gcb, 'BlockFactory', 'com.altera.dspbuilder.blockset.gatecontrol.Multiplexer');  PostSaveFcn=alt_dspbuilder_block_saved(gcb);  NameChangeFcn=alt_dspbuilder_block_renamed(gcb);
      mask Help: helpview(char(com.altera.dspbuilder.simulation.Cache.getBlockTemplate('BlockFactory', 'com.altera.dspbuilder.blockset.gatecontrol.Multiplexer').getHelpFile))
      mask TabNameString: Main,Main,Main,Main,Optional Ports,Optional Ports,Optional Ports,Optional Ports,Optional Ports
      mask Display:
      | port_label('input', 1, 'sel(2:0)');
      | port_label('input', 2, '0-');
      | port_label('input', 3, '1-');
      | port_label('input', 4, '2-');
      | port_label('input', 5, '3-');
      | port_label('input', 6, '4-');
      | port_label('input', 7, '5-');
      | plot([0 0 0.25 1 1 0.25 0], [0 1 1 0.875 0.125 0 0])
      | disp('MUX');
  Multiplier : S-Function  LoadFcn=alt_dspbuilder_load_block(gcb, 'BlockFactory', 'com.altera.dspbuilder.blockset.arithmetic.Multiplier');  FunctionName=sGeneric  Parameters=BusType bwl bwr pipeline pipeline_display allowFloatingPointOverride logOutputs logFile UseEqualInputWidth bbwl bbwr FullResolution OutputMsb OutputLsb OutputBwl OutputBwr UseDedicatedCircuitry use_ena use_aclr  EnableBusSupport=off  mask(Multiplier AlteraBlockset){BusType=Signed Integer, bwl=8, bwr=0, pipeline=0, pipeline_display=0, allowFloatingPointOverride=on, logOutputs=off, logFile=D:\\allblocks%5Falteradspbuilder2_Multiplier.fixedpointlog, UseEqualInputWidth=on, bbwl=8, bbwr=0, FullResolution=on, OutputMsb=8, OutputLsb=0, OutputBwl=16, OutputBwr=16, UseDedicatedCircuitry=YES, use_ena=off, use_aclr=off}
      mask prompts: BusType "Bus Type"; bwl "Input [Number Of Bits].[]"; bwr "Input [].[Number Of Bits]"; pipeline "Number Of Pipeline Stages"; pipeline_display "Number Of Pipeline Stages (Calculated)"; UseEqualInputWidth "Both Inputs Have Same Bit Width"; bbwl "Input b [Number Of Bits].[]"; bbwr "Input b [].[Number Of Bits]"; FullResolution "Full Resolution for Output Result"; OutputMsb "Output MSB"; OutputLsb "Output LSB"; OutputBwl "Output [Number Of Bits].[]"; OutputBwr "Output [].[Number Of Bits]"; UseDedicatedCircuitry "Use Dedicated Circuitry"; use_ena "Use Enable Port (ena)"; use_aclr "Use Asynchronous Clear Port (aclr)"
      mask help:
      | Supports two scalar inputs (no multi-dimensional Simulink signals). Operand a is multiplied by operand b and the result r output as shown by the following equation:
      | r = a x b
      mask init:
      | alt_dspbuilder_init('BlockFactory', 'com.altera.dspbuilder.blockset.arithmetic.Multiplier', { get_param(gcb, 'BusType') bwl bwr pipeline pipeline_display allowFloatingPointOverride logOutputs logFile get_param(gcb, 'UseEqualInputWidth') bbwl bbwr get_param(gcb, 'FullResolution') OutputMsb OutputLsb OutputBwl OutputBwr UseDedicatedCircuitry use_ena use_aclr });
      settings: CopyFcn=alt_dspbuilder_add_block(gcb, 'BlockFactory', 'com.altera.dspbuilder.blockset.arithmetic.Multiplier');  DeleteFcn=com.altera.dspbuilder.simulation.Mask.delete(gcb);  UndoDeleteFcn=alt_dspbuilder_add_block(gcb, 'BlockFactory', 'com.altera.dspbuilder.blockset.arithmetic.Multiplier');  PostSaveFcn=alt_dspbuilder_block_saved(gcb);  NameChangeFcn=alt_dspbuilder_block_renamed(gcb);
      mask Help: helpview(char(com.altera.dspbuilder.simulation.Cache.getBlockTemplate('BlockFactory', 'com.altera.dspbuilder.blockset.arithmetic.Multiplier').getHelpFile))
      mask StyleString: popup(Signed Integer|Unsigned Integer|Signed Fractional|Unsigned Fractional),edit,edit,edit,edit,checkbox,checkbox,edit,checkbox,edit,edit,checkbox,edit,edit,edit,edit,popup(AUTO|YES|NO),checkbox,checkbox
      mask CallbackString: alt_dspbuilder_update_gui('BlockFactory', 'com.altera.dspbuilder.blockset.arithmetic.Multiplier', 'BusType', 0);||||||||alt_dspbuilder_update_gui('BlockFactory', 'com.altera.dspbuilder.blockset.arithmetic.Multiplier', 'UseEqualInputWidth', 8);|||alt_dspbuilder_update_gui('BlockFactory', 'com.altera.dspbuilder.blockset.arithmetic.Multiplier', 'FullResolution', 11);|||||||
      mask TabNameString: Main,Main,Main,Main,Main,Main,Main,Main,Optional Port Sizing,Optional Port Sizing,Optional Port Sizing,Optional Port Sizing,Optional Port Sizing,Optional Port Sizing,Optional Port Sizing,Optional Port Sizing,Optional Ports and Settings,Optional Ports and Settings,Optional Ports and Settings
      mask Display:
      | port_label('input', 1, 'a(7:0)');
      | port_label('input', 2, 'b(7:0)');
      | port_label('output', 1, 'r (15:0)');
      | plot([0 0 0 1 0], [0 1 0 0.5 1])
      | disp('X  ');
  Multiply Accumulate : S-Function  LoadFcn=alt_dspbuilder_load_block(gcb, 'BlockFactory', 'com.altera.dspbuilder.blockset.arithmetic.MultiplyAccumulate');  FunctionName=sGeneric  Parameters=BusType abwl abwr bbwl bbwr ywidth pipeline_register pipeline_display direction use_addsub use_ena use_aclr UseDedicatedCircuitry allowFloatingPointOverride logOutputs logFile  EnableBusSupport=off  mask(MultiplyAccumulate AlteraBlockset){BusType=Signed Integer, abwl=8, abwr=0, bbwl=8, bbwr=0, ywidth=8, pipeline_register=None, pipeline_display=0, direction=Add, use_addsub=off, use_ena=off, use_aclr=off, UseDedicatedCircuitry=YES, allowFloatingPointOverride=on, logOutputs=off, logFile=D:\\allblocks%5Falteradspbuilder2_Multiply+Accumulate.fixedpointlog}
      mask prompts: BusType "Bus Type"; abwl "Input A [Number Of Bits].[]"; abwr "Input A [].[Number Of Bits]"; bbwl "Input B [Number Of Bits].[]"; bbwr "Input B [].[Number Of Bits]"; ywidth "Output Result Number Of Bits"; pipeline_register "Pipeline Register"; pipeline_display "Number Of Pipeline Stages (Calculated)"; direction "Accumulator Direction"; use_addsub "Use Add/Subtract Port (addsub)"; use_ena "Use Enable Port (ena)"; use_aclr "Use Asynchronous Clear Port (aclr)"; UseDedicatedCircuitry "Use Dedicated Multiplier Circuitry"; allowFloatingPointOverride "Allow Floating Point Override For This Block"
      mask help:
      | Consists of a single multiplier feeding an accumulator which performs the calculation:
      |  y += a x b.
      |
      | Note that only 'Data Inputs' and 'Multiplier Output' values for 'Pipeline Register' option will produce the same results for Simulink and HDL simulation for Stratix V, Arria V, Arria V GZ and Cyclone V device families.
      mask init:
      | alt_dspbuilder_init('BlockFactory', 'com.altera.dspbuilder.blockset.arithmetic.MultiplyAccumulate', { get_param(gcb, 'BusType') abwl abwr bbwl bbwr ywidth pipeline_register pipeline_display direction use_addsub use_ena use_aclr UseDedicatedCircuitry allowFloatingPointOverride logOutputs logFile });
      settings: CopyFcn=alt_dspbuilder_add_block(gcb, 'BlockFactory', 'com.altera.dspbuilder.blockset.arithmetic.MultiplyAccumulate');  DeleteFcn=com.altera.dspbuilder.simulation.Mask.delete(gcb);  UndoDeleteFcn=alt_dspbuilder_add_block(gcb, 'BlockFactory', 'com.altera.dspbuilder.blockset.arithmetic.MultiplyAccumulate');  PostSaveFcn=alt_dspbuilder_block_saved(gcb);  NameChangeFcn=alt_dspbuilder_block_renamed(gcb);
      mask Help: helpview(char(com.altera.dspbuilder.simulation.Cache.getBlockTemplate('BlockFactory', 'com.altera.dspbuilder.blockset.arithmetic.MultiplyAccumulate').getHelpFile))
      mask StyleString: popup(Signed Integer|Unsigned Integer|Signed Fractional|Unsigned Fractional),edit,edit,edit,edit,edit,popup(None|Data Inputs|Multiplier Output|Data Inputs and Multiplier),edit,popup(Add|Subtract),checkbox,checkbox,checkbox,popup(AUTO|YES|NO),checkbox,checkbox,edit
      mask CallbackString: alt_dspbuilder_update_gui('BlockFactory', 'com.altera.dspbuilder.blockset.arithmetic.MultiplyAccumulate', 'BusType', 0);|||||||||||||||
      mask TabNameString: Main,Main,Main,Main,Main,Main,Main,Main,Main,Optional Ports and Settings,Optional Ports and Settings,Optional Ports and Settings,Optional Ports and Settings,Optional Ports and Settings,Optional Ports and Settings,Optional Ports and Settings
      mask Display:
      | port_label('input', 1, 'a(7:0)');
      | port_label('input', 2, 'b(7:0)');
      | port_label('input', 3, 'sload');
      | port_label('output', 1, 'y(7:0)');
      | disp('y += a X b');
  Multiply Add : S-Function  LoadFcn=alt_dspbuilder_load_block(gcb, 'BlockFactory', 'com.altera.dspbuilder.blockset.arithmetic.MultiplyAdd');  FunctionName=sGeneric  Parameters=multipliers BusType bwl bwr direction pipeline_register pipeline_display use_constants constants UseDedicatedCircuitry use_ena use_aclr allowFloatingPointOverride logOutputs logFile  EnableBusSupport=off  mask(MultiplyAdd AlteraBlockset){multipliers=2, BusType=Signed Integer, bwl=8, bwr=0, direction=Add Add, pipeline_register=Inputs Multiplier and Adder, pipeline_display=3, use_constants=off, constants=[13 -2 0 3], UseDedicatedCircuitry=on, use_ena=off, use_aclr=off, allowFloatingPointOverride=on, logOutputs=off, logFile=D:\\allblocks%5Falteradspbuilder2_Multiply+Add.fixedpointlog}
      mask prompts: multipliers "Number Of Multipliers (2-4)"; BusType "Bus Type"; bwl "Input [Number Of Bits].[]"; bwr "Input [].[Number Of Bits]"; direction "Adder Mode"; pipeline_register "Pipeline Register"; pipeline_display "Number Of Pipeline Stages (Calculated)"; use_constants "One Input is Constant"; constants "Constant Values"; UseDedicatedCircuitry "Use Dedicated Circuitry"; use_ena "Use Enable Port (ena)"; use_aclr "Use Asynchronous Clear Port (aclr)"; allowFloatingPointOverride "Allow Floating Point Override For This Block"
      mask help:
      | Consists of two, three, or four multipliers feeding a parallel adder. The operands in each pair are multiplied together and the second and fourth multiplier outputs can optionally be added to or subtracted from the total.
      |
      | The block function can be expressed by the equation:
      |  y = a0xb0 +/- a1xb1 [+ a2xb2 [+/- a3xb3]]]
      |
      | The operand b inputs can optionally be hidden and instead have constant values assigned to them.
      |
      | Pipeline Register options that include 'Multiplier' are not available on Stratix V, Arria V or Cyclone V.
      mask init:
      | alt_dspbuilder_init('BlockFactory', 'com.altera.dspbuilder.blockset.arithmetic.MultiplyAdd', { get_param(gcb, 'multipliers') get_param(gcb, 'BusType') bwl bwr get_param(gcb, 'direction') get_param(gcb, 'pipeline_register') pipeline_display get_param(gcb, 'use_constants') constants UseDedicatedCircuitry get_param(gcb, 'use_ena') get_param(gcb, 'use_aclr') allowFloatingPointOverride logOutputs logFile });
      settings: CopyFcn=alt_dspbuilder_add_block(gcb, 'BlockFactory', 'com.altera.dspbuilder.blockset.arithmetic.MultiplyAdd');  DeleteFcn=com.altera.dspbuilder.simulation.Mask.delete(gcb);  UndoDeleteFcn=alt_dspbuilder_add_block(gcb, 'BlockFactory', 'com.altera.dspbuilder.blockset.arithmetic.MultiplyAdd');  PostSaveFcn=alt_dspbuilder_block_saved(gcb);  NameChangeFcn=alt_dspbuilder_block_renamed(gcb);
      mask Help: helpview(char(com.altera.dspbuilder.simulation.Cache.getBlockTemplate('BlockFactory', 'com.altera.dspbuilder.blockset.arithmetic.MultiplyAdd').getHelpFile))
      mask StyleString: popup(2|3|4),popup(Signed Integer|Unsigned Integer|Signed Fractional|Unsigned Fractional),edit,edit,popup(Add Add|Add Sub|Sub Add|Sub Sub),popup(No Register|Inputs Only|Multiplier Only|Adder Only|Inputs and Multiplier|Inputs and Adder|Multiplier and Adder|Inputs Multiplier and Adder),edit,checkbox,edit,checkbox,checkbox,checkbox,checkbox,checkbox,edit
      mask CallbackString: alt_dspbuilder_update_gui('BlockFactory', 'com.altera.dspbuilder.blockset.arithmetic.MultiplyAdd', 'multipliers', 0);|alt_dspbuilder_update_gui('BlockFactory', 'com.altera.dspbuilder.blockset.arithmetic.MultiplyAdd', 'BusType', 1);|||alt_dspbuilder_update_gui('BlockFactory', 'com.altera.dspbuilder.blockset.arithmetic.MultiplyAdd', 'direction', 4);|alt_dspbuilder_update_gui('BlockFactory', 'com.altera.dspbuilder.blockset.arithmetic.MultiplyAdd', 'pipeline_register', 5);||alt_dspbuilder_update_gui('BlockFactory', 'com.altera.dspbuilder.blockset.arithmetic.MultiplyAdd', 'use_constants', 7);|||alt_dspbuilder_update_gui('BlockFactory', 'com.altera.dspbuilder.blockset.arithmetic.MultiplyAdd', 'use_ena', 10);|alt_dspbuilder_update_gui('BlockFactory', 'com.altera.dspbuilder.blockset.arithmetic.MultiplyAdd', 'use_aclr', 11);|||
      mask TabNameString: Main,Main,Main,Main,Main,Main,Main,Optional Ports and Settings,Optional Ports and Settings,Optional Ports and Settings,Optional Ports and Settings,Optional Ports and Settings,Optional Ports and Settings,Optional Ports and Settings,Optional Ports and Settings
      mask Display:
      | port_label('input', 1, 'a0(7:0)');
      | port_label('input', 2, 'b0(7:0)');
      | port_label('input', 3, 'a1(7:0)');
      | port_label('input', 4, 'b1(7:0)');
      | port_label('output', 1, 'y(16:0)');
      | disp('y = a0 X b0 + a1 X b1');
  Non-synthesizable Input : S-Function  LoadFcn=alt_dspbuilder_load_block(gcb, 'BlockFactory', 'com.altera.dspbuilder.blockset.iobus.NonSynthInput');  FunctionName=sInOut  Parameters=iofile BusType bwl bwr SpecifyClock allowFloatingPointOverride logOutputs externalType  EnableBusSupport=off  mask(Non-synthesizable Input AlteraBlockset){iofile=, BusType=Signed Integer, bwl=8, bwr=0, SpecifyClock=off, clock=, allowFloatingPointOverride=on, logOutputs=off, externalType=Inferred}
      mask prompts: BusType "Bus Type"; bwl "[Number Of Bits].[]"; bwr "[].[Number Of Bits]"; SpecifyClock "Specify Clock"; allowFloatingPointOverride "Allow Floating Point Override For This Block"; externalType "External Type"
      mask help:
      | Marks an entry point to a non-synthesizable DSP Builder system.
      |
      | Because DSP Builder registers its own type with Simulink, this block is necessary to use the DSP Builder blocks when they are not intended to be synthesized as part of the final design. This block should be used in conjunction with a Non-Synthesizable Output block to mark the exit point from the system.
      mask init:
      | alt_dspbuilder_init_io('BlockFactory', 'com.altera.dspbuilder.blockset.iobus.NonSynthInput', { iofile get_param(gcb, 'BusType') bwl bwr get_param(gcb, 'SpecifyClock') clock allowFloatingPointOverride logOutputs externalType });
      settings: CopyFcn=alt_dspbuilder_add_block(gcb, 'BlockFactory', 'com.altera.dspbuilder.blockset.iobus.NonSynthInput');  DeleteFcn=com.altera.dspbuilder.simulation.Mask.delete(gcb);  UndoDeleteFcn=alt_dspbuilder_add_block(gcb, 'BlockFactory', 'com.altera.dspbuilder.blockset.iobus.NonSynthInput');  PostSaveFcn=alt_dspbuilder_block_saved(gcb);  NameChangeFcn=alt_dspbuilder_block_renamed(gcb);
      mask Help: helpview(char(com.altera.dspbuilder.simulation.Cache.getBlockTemplate('BlockFactory', 'com.altera.dspbuilder.blockset.iobus.NonSynthInput').getHelpFile))
      mask StyleString: edit,popup(Signed Integer|Unsigned Integer|Signed Fractional|Unsigned Fractional|Single Bit),edit,edit,checkbox,edit,checkbox,checkbox,popup(Inferred|Simulink Fixed Point Type|Double)
      mask CallbackString: |alt_dspbuilder_update_gui('BlockFactory', 'com.altera.dspbuilder.blockset.iobus.NonSynthInput', 'BusType', 1);|||alt_dspbuilder_update_gui('BlockFactory', 'com.altera.dspbuilder.blockset.iobus.NonSynthInput', 'SpecifyClock', 4);||||
      mask Display:
      | plot([ [ 15 -15] -(15 + 5 * sin(0:0.1:pi)) [ -15 15 20  15] ], [ [-10 -10]       -10 * cos(0:0.1:pi) [ 10  10  0 -10] ])
      | plot([ [ 13 -13] -(13 + 5 * sin(0:0.1:pi)) [ -13 13 18  13] ], [ [-10 -10]       -10 * cos(0:0.1:pi) [ 10  10  0 -10] ])
      | disp('i7:0')
  Non-synthesizable Output : S-Function  LoadFcn=alt_dspbuilder_load_block(gcb, 'BlockFactory', 'com.altera.dspbuilder.blockset.iobus.NonSynthOutput');  FunctionName=sInOut  Parameters=iofile BusType bwl bwr allowFloatingPointOverride logOutputs externalType  EnableBusSupport=off  mask(Non-synthesizable Output AlteraBlockset){iofile=, BusType=Signed Integer, bwl=8, bwr=0, allowFloatingPointOverride=on, logOutputs=off, externalType=Inferred}
      mask prompts: BusType "Bus Type"; bwl "[Number Of Bits].[]"; bwr "[].[Number Of Bits]"; allowFloatingPointOverride "Allow Floating Point Override For This Block"; externalType "External Type"
      mask help:
      | Marks an exit point from a non-synthesizable DSP Builder system.
      |
      | Because DSP Builder registers its own type with Simulink, this block is necessary to use the DSP Builder blocks when they are not intended to be synthesized as part of the final design. This block should be used in conjunction with the Non-Synthesizable
      | Input block to mark the entry point. You can also use this block to create a non-synthesizable output from a synthesizable system.
      mask init:
      | alt_dspbuilder_init_io('BlockFactory', 'com.altera.dspbuilder.blockset.iobus.NonSynthOutput', { iofile get_param(gcb, 'BusType') bwl bwr allowFloatingPointOverride logOutputs externalType });
      settings: CopyFcn=alt_dspbuilder_add_block(gcb, 'BlockFactory', 'com.altera.dspbuilder.blockset.iobus.NonSynthOutput');  DeleteFcn=com.altera.dspbuilder.simulation.Mask.delete(gcb);  UndoDeleteFcn=alt_dspbuilder_add_block(gcb, 'BlockFactory', 'com.altera.dspbuilder.blockset.iobus.NonSynthOutput');  PostSaveFcn=alt_dspbuilder_block_saved(gcb);  NameChangeFcn=alt_dspbuilder_block_renamed(gcb);
      mask Help: helpview(char(com.altera.dspbuilder.simulation.Cache.getBlockTemplate('BlockFactory', 'com.altera.dspbuilder.blockset.iobus.NonSynthOutput').getHelpFile))
      mask StyleString: edit,popup(Inferred|Signed Integer|Unsigned Integer|Signed Fractional|Unsigned Fractional|Single Bit),edit,edit,checkbox,checkbox,popup(Inferred|Simulink Fixed Point Type|Double)
      mask CallbackString: |alt_dspbuilder_update_gui('BlockFactory', 'com.altera.dspbuilder.blockset.iobus.NonSynthOutput', 'BusType', 1);|||||
      mask Display:
      | plot([ [ 15 -15 -20 -15 15] (15 + 5 * sin(0:0.1:pi))], [ [-10 -10   0  10 10]       10 * cos(0:0.1:pi)])
      | plot([ [ 13 -13 -18 -13 13] (13 + 5 * sin(0:0.1:pi))], [ [-10 -10   0  10 10]       10 * cos(0:0.1:pi)])
      | disp('o7:0')
  Output : S-Function  LoadFcn=alt_dspbuilder_load_block(gcb, 'BlockFactory', 'com.altera.dspbuilder.blockset.iobus.Output');  FunctionName=sInOut  Parameters=iofile BusType bwl bwr externalType allowFloatingPointOverride logOutputs  EnableBusSupport=off  mask(Output AlteraBlockset){iofile=d:\\SJ\\nightly\\13.1\\162\\w32\\acds\\quartus\\dsp_builder\\bin\\mdllibrary\\tb_allblocks_alteradspbuilder2\\allblocks%5Falteradspbuilder2_Output.capture, BusType=Signed Integer, bwl=8, bwr=0, externalType=Inferred, PORTTYPE=Output, allowFloatingPointOverride=on, logOutputs=off}
      mask prompts: BusType "Bus Type"; bwl "[Number Of Bits].[]"; bwr "[].[Number Of Bits]"; externalType "External Type"; PORTTYPE "TYPE"; allowFloatingPointOverride "Allow Floating Point Override For This Block"
      mask help:
      | Defines the output boundary of a hardware system and casts signed binary fractional format (from DSP Builder blocks) to floating-point Simulink signals (feeding generic Simulink blocks).
      |
      | In simulation, this block casts a DSP Builder internal signal to a Simulink signal. You can choose from signed integer, unsigned integer, signed fractional representation or allow the type to be inferred from the previous block.
      |
      | Output blocks map to output ports in VHDL and mark the edge of the generated system. You would normally connect these blocks to Simulink simulation blocks in your testbench. Their outputs should not be connected to other Altera blocks.
      mask init:
      | alt_dspbuilder_init_io('BlockFactory', 'com.altera.dspbuilder.blockset.iobus.Output', { iofile get_param(gcb, 'BusType') bwl bwr externalType PORTTYPE allowFloatingPointOverride logOutputs });
      settings: CopyFcn=alt_dspbuilder_add_block(gcb, 'BlockFactory', 'com.altera.dspbuilder.blockset.iobus.Output');  DeleteFcn=com.altera.dspbuilder.simulation.Mask.delete(gcb);  UndoDeleteFcn=alt_dspbuilder_add_block(gcb, 'BlockFactory', 'com.altera.dspbuilder.blockset.iobus.Output');  PreSaveFcn=alt_dspbuilder_internal_presave_block(gcb);  PostSaveFcn=alt_dspbuilder_block_saved(gcb);  NameChangeFcn=alt_dspbuilder_block_renamed(gcb);
      mask Help: helpview(char(com.altera.dspbuilder.simulation.Cache.getBlockTemplate('BlockFactory', 'com.altera.dspbuilder.blockset.iobus.Output').getHelpFile))
      mask StyleString: edit,popup(Inferred|Signed Integer|Unsigned Integer|Signed Fractional|Unsigned Fractional|Single Bit),edit,edit,popup(Inferred|Simulink Fixed Point Type|Double),edit,checkbox,checkbox
      mask CallbackString: |alt_dspbuilder_update_gui('BlockFactory', 'com.altera.dspbuilder.blockset.iobus.Output', 'BusType', 1);||||||
      mask Display:
      | plot([-25 15 25 15 -25 -25]*-1, [0 0 -10 -20 -20 0] - 0);
      | plot([11 21 11]*-1, [0 -10 -20] - 0);
      | text(0, -10, 'o7:0', 'horizontalAlignment','center','verticalAlignment','middle');
  PLL : S-Function  LoadFcn=|  InitFcn=alt_dspbuilder_internal_initfcn_pll(gcb);  FunctionName=sNoOp  Parameters=clock_mult clock_divide clock_export num_clocks input_clock use_base_clock  EnableBusSupport=off  mask(PLL AlteraBlockset){clock_mult=[1], clock_divide=[1], clock_export=[0], num_clocks=1, input_clock=, use_base_clock=on}
      | alt_dspbuilder_load_block(gcb, 'BlockFactory', 'com.altera.dspbuilder.blockset.RateChange.PLL');
      | alt_dspbuilder_load_clock(gcb, 'BlockFactory', 'com.altera.dspbuilder.blockset.RateChange.PLL');
      mask prompts: clock_mult "Clock Multipliers"; clock_divide "Clock Dividers"; clock_export "Clock Export Values"; num_clocks "Number of Output Clocks"; input_clock "Input Clock"; use_base_clock "Use Base Clock"
      mask help:
      | Generates internal clocks with frequencies that are multiples of the frequency of the system clock on the input clock pin.
      |
      | If you use a PLL block to define clock signals when there is no Clock block in your design, the PLL-derived clocks might not pass the derived period correctly to the blocks referencing the PLL-derived clock. Always explicitly include a Clock block when using a PLL block.
      mask init:
      | alt_dspbuilder_init('BlockFactory', 'com.altera.dspbuilder.blockset.RateChange.PLL', { clock_mult clock_divide clock_export num_clocks input_clock use_base_clock });
      settings: CopyFcn=alt_dspbuilder_add_block(gcb, 'BlockFactory', 'com.altera.dspbuilder.blockset.RateChange.PLL');  DeleteFcn=com.altera.dspbuilder.simulation.Mask.delete(gcb);  UndoDeleteFcn=alt_dspbuilder_add_block(gcb, 'BlockFactory', 'com.altera.dspbuilder.blockset.RateChange.PLL');  PostSaveFcn=alt_dspbuilder_block_saved(gcb);  NameChangeFcn=alt_dspbuilder_block_renamed(gcb);
      settings: OpenFcn=|
      | com.altera.dspbuilder.simulation.Mask.simpleInit('BlockFactory', 'com.altera.dspbuilder.blockset.RateChange.PLL', bdroot(gcb), gcb);
      | alt_PllLaunch(gcb)
      mask Help: helpview(char(com.altera.dspbuilder.simulation.Cache.getBlockTemplate('BlockFactory', 'com.altera.dspbuilder.blockset.RateChange.PLL').getHelpFile))
      mask Display: plot([0 0 1 1 2 2 3 3 4],[0 1 1 0 0 1 1 0 0]);
  Parallel Adder Subtractor : S-Function  LoadFcn=alt_dspbuilder_load_block(gcb, 'BlockFactory', 'com.altera.dspbuilder.blockset.arithmetic.ParallelAdder');  FunctionName=sGeneric  Parameters=number_of_inputs direction use_pipeline pipeline_display phase_selection use_ena use_aclr allowFloatingPointOverride logOutputs logFile  EnableBusSupport=off  mask(ParallelAdder AlteraBlockset){number_of_inputs=4, direction=+, use_pipeline=on, pipeline_display=2, phase_selection=1, use_ena=off, use_aclr=off, allowFloatingPointOverride=on, logOutputs=off, logFile=D:\\allblocks%5Falteradspbuilder2_Parallel+Adder+Subtractor.fixedpointlog}
      mask prompts: number_of_inputs "Number of Inputs"; direction "Add (+) Sub (-)"; use_pipeline "Enable Pipeline (variable length)"; pipeline_display "Number Of Pipeline Stages (Calculated)"; phase_selection "Clock Phase Selection"; use_ena "Use Enable Port (ena)"; use_aclr "Use Asynchronous Clear Port (aclr)"; allowFloatingPointOverride "Allow Floating Point Override For This Block"
      mask help:
      | Adds or subtracts a variable number of input wires. The number of inputs determines the number of input wires to combine.
      |
      | Add (+) Sub (-) is a string of + and - operators determining whether each input is added to or subtracted from the total. Each consecutive pair can be ++, +- or -+, but -- is not legal. Missing symbols are assumed to be + operators.
      |
      | Enable Pipeline registers the output of each stage of the adder tree; this results in a total pipeline of length:
      |  ceil(log2(number of inputs)).
      |
      | Clock Phase Selection is a binary string which sets the phases in which the block is enabled. This is ignored if the pipeline is disabled.
      |
      | The optional enable and asynchronous clear ports allow the pipeline to be paused and cleared.
      mask init:
      | alt_dspbuilder_init('BlockFactory', 'com.altera.dspbuilder.blockset.arithmetic.ParallelAdder', { number_of_inputs direction get_param(gcb, 'use_pipeline') pipeline_display phase_selection use_ena use_aclr allowFloatingPointOverride logOutputs logFile });
      settings: CopyFcn=alt_dspbuilder_add_block(gcb, 'BlockFactory', 'com.altera.dspbuilder.blockset.arithmetic.ParallelAdder');  DeleteFcn=com.altera.dspbuilder.simulation.Mask.delete(gcb);  UndoDeleteFcn=alt_dspbuilder_add_block(gcb, 'BlockFactory', 'com.altera.dspbuilder.blockset.arithmetic.ParallelAdder');  PostSaveFcn=alt_dspbuilder_block_saved(gcb);  NameChangeFcn=alt_dspbuilder_block_renamed(gcb);
      mask Help: helpview(char(com.altera.dspbuilder.simulation.Cache.getBlockTemplate('BlockFactory', 'com.altera.dspbuilder.blockset.arithmetic.ParallelAdder').getHelpFile))
      mask CallbackString: ||alt_dspbuilder_update_gui('BlockFactory', 'com.altera.dspbuilder.blockset.arithmetic.ParallelAdder', 'use_pipeline', 2);|||||||
      mask TabNameString: Main,Main,Main,Main,Optional Ports,Optional Ports,Optional Ports,Optional Ports,Optional Ports,Optional Ports
      mask Display:
      | port_label('input', 1, '+');
      | port_label('input', 2, '+');
      | port_label('input', 3, '+');
      | port_label('input', 4, '+');
      | port_label('output', 1, 'r');
      | plot([-i +i -exp((pi/2:.02*pi:1.5*pi)*i)])
      | disp('+');
  Parallel To Serial : S-Function  LoadFcn=alt_dspbuilder_load_block(gcb, 'BlockFactory', 'com.altera.dspbuilder.blockset.storage.ParallelToSerial');  FunctionName=sGeneric  Parameters=BusType bwl bwr msbfirsttext msbfirst repeatlastbit use_ena use_sclr  EnableBusSupport=off  mask(Parallel To Serial AlteraBlockset){BusType=Signed Integer, bwl=8, bwr=0, msbfirsttext=MSB First, msbfirst=1, repeatlastbit=on, use_ena=on, use_sclr=off}
      mask prompts: BusType "Data Bus Type"; bwl "[Number Of Bits].[]"; bwr "[].[Number Of Bits]"; msbfirsttext "Serial Bit Order"; msbfirst "Serial Bit Order Boolean"; repeatlastbit "Repeat Last Bit Until Next Load"; use_ena "Use Enable Port (ena)"; use_sclr "Use Synchronous Clear port (sclr)"
      mask help:
      | Implements a parallel (input d) to serial bus conversion (output sd).
      |
      | The output bit stream can be created as either Most Significant Bit (MSB) first, or Least Significant Bit (LSB) first.
      mask init:
      | alt_dspbuilder_init('BlockFactory', 'com.altera.dspbuilder.blockset.storage.ParallelToSerial', { get_param(gcb, 'BusType') bwl bwr msbfirsttext msbfirst repeatlastbit use_ena use_sclr });
      settings: CopyFcn=alt_dspbuilder_add_block(gcb, 'BlockFactory', 'com.altera.dspbuilder.blockset.storage.ParallelToSerial');  DeleteFcn=com.altera.dspbuilder.simulation.Mask.delete(gcb);  UndoDeleteFcn=alt_dspbuilder_add_block(gcb, 'BlockFactory', 'com.altera.dspbuilder.blockset.storage.ParallelToSerial');  PostSaveFcn=alt_dspbuilder_block_saved(gcb);  NameChangeFcn=alt_dspbuilder_block_renamed(gcb);
      mask Help: helpview(char(com.altera.dspbuilder.simulation.Cache.getBlockTemplate('BlockFactory', 'com.altera.dspbuilder.blockset.storage.ParallelToSerial').getHelpFile))
      mask StyleString: popup(Signed Integer|Unsigned Integer|Signed Fractional|Unsigned Fractional),edit,edit,popup(MSB First|LSB First),edit,checkbox,checkbox,checkbox
      mask CallbackString: alt_dspbuilder_update_gui('BlockFactory', 'com.altera.dspbuilder.blockset.storage.ParallelToSerial', 'BusType', 0);|||||||
      mask TabNameString: Main,Main,Main,Main,Main,Main,Optional Ports,Optional Ports
      mask Display:
      | port_label('input', 1, 'd(7:0)');
      | port_label('input', 2, 'ena');
      | port_label('input', 3, 'load');
      | port_label('output', 1, 'sd');
  Pattern : S-Function  LoadFcn=alt_dspbuilder_load_block(gcb, 'BlockFactory', 'com.altera.dspbuilder.blockset.gatecontrol.Pattern');  FunctionName=sGeneric  Parameters=Sequence SpecifyClock use_ena use_sclr  EnableBusSupport=off  mask(Pattern AlteraBlockset){Sequence=100000, SpecifyClock=off, clock=, use_ena=off, use_sclr=off}
      mask prompts: Sequence "Binary Sequence"; SpecifyClock "Specify Clock"; use_ena "Use Enable Port (ena)"; use_sclr "Use Synchronous Clear Port (sclr)"
      mask help:
      | Generates a repeating periodic bit sequence in time. You can enter the required pattern as a binary sequence using '1' and '0' only. The output starts from the left of the sequence.
      |
      | For example, 1000, outputs a '1' followed by four '0@ and repeats this sequence every four samples.
      |
      | Note: When used with a sequence of length 1 this block acts as a constant, holding its output at the specified value at all times.
      mask init:
      | alt_dspbuilder_init('BlockFactory', 'com.altera.dspbuilder.blockset.gatecontrol.Pattern', { Sequence get_param(gcb, 'SpecifyClock') clock use_ena use_sclr });
      settings: CopyFcn=alt_dspbuilder_add_block(gcb, 'BlockFactory', 'com.altera.dspbuilder.blockset.gatecontrol.Pattern');  DeleteFcn=com.altera.dspbuilder.simulation.Mask.delete(gcb);  UndoDeleteFcn=alt_dspbuilder_add_block(gcb, 'BlockFactory', 'com.altera.dspbuilder.blockset.gatecontrol.Pattern');  PostSaveFcn=alt_dspbuilder_block_saved(gcb);  NameChangeFcn=alt_dspbuilder_block_renamed(gcb);
      mask Help: helpview(char(com.altera.dspbuilder.simulation.Cache.getBlockTemplate('BlockFactory', 'com.altera.dspbuilder.blockset.gatecontrol.Pattern').getHelpFile))
      mask CallbackString: |alt_dspbuilder_update_gui('BlockFactory', 'com.altera.dspbuilder.blockset.gatecontrol.Pattern', 'SpecifyClock', 1);|||
      mask TabNameString: Main,Main,Main,Optional Ports,Optional Ports
      mask Display: disp(Sequence);
  Pipelined Adder : S-Function  LoadFcn=alt_dspbuilder_load_block(gcb, 'BlockFactory', 'com.altera.dspbuilder.blockset.arithmetic.PipelinedAdder');  FunctionName=sGeneric  Parameters=BusType bwl bwr pipeline pipeline_display AddSubDirection use_cin use_ovl use_addsub use_ena use_aclr or_aclr_inputs  EnableBusSupport=off  mask(Pipelined Adder AlteraBlockset){BusType=Signed Integer, bwl=8, bwr=0, pipeline=2, pipeline_display=2, AddSubDirection=ADD, use_cin=off, use_ovl=off, use_addsub=off, use_ena=off, use_aclr=off, or_aclr_inputs=on}
      mask prompts: BusType "Bus Type"; bwl "[Number Of Bits].[]"; bwr "[].[Number Of Bits]"; pipeline "Number of Pipeline Stages"; pipeline_display "Number Of Pipeline Stages (Calculated)"; AddSubDirection "Direction"; use_cin "Use Carry In Port (cin)"; use_ovl "Use Overflow/Carry Out port (ovl)"; use_addsub "Use Direction Port (addsub)"; use_ena "Use Enable Port (ena)"; use_aclr "Use Asynchronous Clear Port (aclr)"; or_aclr_inputs "'OR' Asynchronous Clear Input with Global Aclr"
      mask help:
      | Performs the following calculation:
      |  r = a + b + cin when adding (addsub = 1)
      |  r = a - b + cin -1 when subtracting (addsub = 0)
      |
      | The optional ovl port is used as an overflow when using signed arithmetic or as a carry out when using unsigned arithmetic. In the case of unsigned subtraction, this means the output is 1 when no overflow has occurred.
      mask init:
      | alt_dspbuilder_init('BlockFactory', 'com.altera.dspbuilder.blockset.arithmetic.PipelinedAdder', { get_param(gcb, 'BusType') bwl bwr pipeline pipeline_display AddSubDirection use_cin use_ovl get_param(gcb, 'use_addsub') use_ena get_param(gcb, 'use_aclr') get_param(gcb, 'or_aclr_inputs') });
      settings: CopyFcn=alt_dspbuilder_add_block(gcb, 'BlockFactory', 'com.altera.dspbuilder.blockset.arithmetic.PipelinedAdder');  DeleteFcn=com.altera.dspbuilder.simulation.Mask.delete(gcb);  UndoDeleteFcn=alt_dspbuilder_add_block(gcb, 'BlockFactory', 'com.altera.dspbuilder.blockset.arithmetic.PipelinedAdder');  PostSaveFcn=alt_dspbuilder_block_saved(gcb);  NameChangeFcn=alt_dspbuilder_block_renamed(gcb);
      mask Help: helpview(char(com.altera.dspbuilder.simulation.Cache.getBlockTemplate('BlockFactory', 'com.altera.dspbuilder.blockset.arithmetic.PipelinedAdder').getHelpFile))
      mask StyleString: popup(Inferred|Signed Integer|Unsigned Integer|Signed Fractional|Unsigned Fractional),edit,edit,edit,edit,popup(ADD|SUB),checkbox,checkbox,checkbox,checkbox,checkbox,checkbox
      mask CallbackString: alt_dspbuilder_update_gui('BlockFactory', 'com.altera.dspbuilder.blockset.arithmetic.PipelinedAdder', 'BusType', 0);||||||||alt_dspbuilder_update_gui('BlockFactory', 'com.altera.dspbuilder.blockset.arithmetic.PipelinedAdder', 'use_addsub', 8);||alt_dspbuilder_update_gui('BlockFactory', 'com.altera.dspbuilder.blockset.arithmetic.PipelinedAdder', 'use_aclr', 10);|alt_dspbuilder_update_gui('BlockFactory', 'com.altera.dspbuilder.blockset.arithmetic.PipelinedAdder', 'or_aclr_inputs', 11);
      mask TabNameString: Main,Main,Main,Main,Main,Optional Ports and Settings,Optional Ports and Settings,Optional Ports and Settings,Optional Ports and Settings,Optional Ports and Settings,Optional Ports and Settings,Optional Ports and Settings
      mask Display:
      | port_label('input', 1, 'a');
      | port_label('input', 2, 'b');
      | port_label('output', 1, 'r');
      | plot([-i +i -exp((pi/2:.02*pi:1.5*pi)*i)])
      | disp('+');
  Product : S-Function  LoadFcn=alt_dspbuilder_load_block(gcb, 'BlockFactory', 'com.altera.dspbuilder.blockset.arithmetic.Product');  FunctionName=sGeneric  Parameters=BusType bwl bwr pipeline pipeline_display phase_selection use_ena use_aclr UseLPM UseDedicatedCircuitry allowFloatingPointOverride logOutputs logFile  EnableBusSupport=off  mask(Product AlteraBlockset){BusType=Inferred, bwl=8, bwr=0, pipeline=0, pipeline_display=0, phase_selection=1, use_ena=off, use_aclr=off, UseLPM=off, UseDedicatedCircuitry=on, allowFloatingPointOverride=on, logOutputs=off, logFile=D:\\allblocks%5Falteradspbuilder2_Product.fixedpointlog}
      mask prompts: BusType "Bus Type"; bwl "[Number Of Bits].[]"; bwr "[].[Number Of Bits]"; pipeline "Number of Pipeline Stages"; pipeline_display "Number Of Pipeline Stages (Calculated)"; phase_selection "Clock Phase Selection"; use_ena "Use Enable Port (ena)"; use_aclr "Use Asynchronous Clear Port (aclr)"; UseLPM "Use LPM"; UseDedicatedCircuitry "Use Dedicated Circuitry"; allowFloatingPointOverride "Allow Floating Point Override For This Block"
      mask help:
      | Supports two scalar inputs (no multi-dimensional Simulink signals). Operand a is multiplied by operand b and the result output on r as shown by the following equation:
      |  r = a x b
      mask init:
      | alt_dspbuilder_init('BlockFactory', 'com.altera.dspbuilder.blockset.arithmetic.Product', { get_param(gcb, 'BusType') bwl bwr pipeline pipeline_display phase_selection use_ena use_aclr UseLPM UseDedicatedCircuitry allowFloatingPointOverride logOutputs logFile });
      settings: CopyFcn=alt_dspbuilder_add_block(gcb, 'BlockFactory', 'com.altera.dspbuilder.blockset.arithmetic.Product');  DeleteFcn=com.altera.dspbuilder.simulation.Mask.delete(gcb);  UndoDeleteFcn=alt_dspbuilder_add_block(gcb, 'BlockFactory', 'com.altera.dspbuilder.blockset.arithmetic.Product');  PostSaveFcn=alt_dspbuilder_block_saved(gcb);  NameChangeFcn=alt_dspbuilder_block_renamed(gcb);
      mask Help: helpview(char(com.altera.dspbuilder.simulation.Cache.getBlockTemplate('BlockFactory', 'com.altera.dspbuilder.blockset.arithmetic.Product').getHelpFile))
      mask StyleString: popup(Inferred|Signed Integer|Unsigned Integer|Signed Fractional|Unsigned Fractional),edit,edit,edit,edit,edit,checkbox,checkbox,checkbox,checkbox,checkbox,checkbox,edit
      mask CallbackString: alt_dspbuilder_update_gui('BlockFactory', 'com.altera.dspbuilder.blockset.arithmetic.Product', 'BusType', 0);||||||||||||
      mask TabNameString: Main,Main,Main,Main,Main,Optional Ports and Settings,Optional Ports and Settings,Optional Ports and Settings,Optional Ports and Settings,Optional Ports and Settings,Optional Ports and Settings,Optional Ports and Settings,Optional Ports and Settings
      mask Display:
      | port_label('input', 1, 'a');
      | port_label('input', 2, 'b');
      | port_label('output', 1, 'r  ');
      | plot([0 0 0 1 0], [0 1 0 0.5 1])
      | disp('X  ');
  Quartus II Global Project Assignments : S-Function  LoadFcn=alt_dspbuilder_load_block(gcb, 'BlockFactory', 'com.altera.dspbuilder.blockset.altlab.QuartusIIGlobalAssignment');  FunctionName=sNoOp  Parameters=QuartusIIAssignmentName QuartusIIAssignmentValue  EnableBusSupport=off  mask(Quartus II Global Project Assignments AlteraBlockset){QuartusIIAssignmentName=, QuartusIIAssignmentValue=}
      mask prompts: QuartusIIAssignmentName "Assignment Name"; QuartusIIAssignmentValue "Assignment Value"
      mask help:
      | Passes Quartus II project global assignments to the Quartus II project generated by the Signal Compiler block.
      |
      | Each block sets a single assignment, but multiple blocks can be used for multiple assignments.
      |
      | A full list of possible assignments is given in the Quartus II Settings File Reference Manual.
      |
      | Illegal or unrecognized assignments are detected during Signal Compiler Quartus II project generation, and result in a failure to create the Quartus II project.
      mask init:
      | alt_dspbuilder_init('BlockFactory', 'com.altera.dspbuilder.blockset.altlab.QuartusIIGlobalAssignment', { QuartusIIAssignmentName QuartusIIAssignmentValue });
      settings: CopyFcn=alt_dspbuilder_add_block(gcb, 'BlockFactory', 'com.altera.dspbuilder.blockset.altlab.QuartusIIGlobalAssignment');  DeleteFcn=com.altera.dspbuilder.simulation.Mask.delete(gcb);  UndoDeleteFcn=alt_dspbuilder_add_block(gcb, 'BlockFactory', 'com.altera.dspbuilder.blockset.altlab.QuartusIIGlobalAssignment');  PostSaveFcn=alt_dspbuilder_block_saved(gcb);  NameChangeFcn=alt_dspbuilder_block_renamed(gcb);
      mask Help: helpview(char(com.altera.dspbuilder.simulation.Cache.getBlockTemplate('BlockFactory', 'com.altera.dspbuilder.blockset.altlab.QuartusIIGlobalAssignment').getHelpFile))
      mask Display:
      | plot([0 0 9 10 9 9 10 10 0],[0 10 10 7 7 10 7 0 0]);
      | fprintf('%s\n%s', QuartusIIAssignmentName, QuartusIIAssignmentValue);
  Quartus II Pinout Assignments : S-Function  LoadFcn=alt_dspbuilder_load_block(gcb, 'BlockFactory', 'com.altera.dspbuilder.blockset.altlab.QuartusIIPinAssignment');  FunctionName=sNoOp  Parameters=QuartusIIAssignmentName QuartusIIAssignmentValue  EnableBusSupport=off  mask(Quartus II Pinout Assignments AlteraBlockset){QuartusIIAssignmentName=, QuartusIIAssignmentValue=}
      mask prompts: QuartusIIAssignmentName "Pin Name"; QuartusIIAssignmentValue "Pin Location"
      mask help:
      | Sets pinout assignments for the Input and Output blocks at the top level of your design.
      | This block can only be used at the top level of the model.
      |
      | The pin names must be the exact instance names of the Input or Output blocks.
      |
      | For busses, use a comma to separate the bit pin assignment location from LSB to MSB.
      | For example:
      |   Pin name : abc
      |   Pin location : Pin_AA, Pin_AB, Pin_AC
      |   assigns abc[0] to Pin_AA, abc[1] to Pin_AB, and abc[2] to Pin_AC
      |
      | To set the pin assignment of the implicit hardware system clock, use the name of the Clock block for the pin name.
      | For example:
      |    Pin name : clock
      |    Pin location : Pin_AM17
      |
      | To set the pin assignment of the implicit hardware global reset, use 'sclr' for the pin name.
      | For example:
      |    Pin name : sclr
      |    Pin location : Pin_B4
      mask init:
      | alt_dspbuilder_init('BlockFactory', 'com.altera.dspbuilder.blockset.altlab.QuartusIIPinAssignment', { QuartusIIAssignmentName QuartusIIAssignmentValue });
      settings: CopyFcn=alt_dspbuilder_add_block(gcb, 'BlockFactory', 'com.altera.dspbuilder.blockset.altlab.QuartusIIPinAssignment');  DeleteFcn=com.altera.dspbuilder.simulation.Mask.delete(gcb);  UndoDeleteFcn=alt_dspbuilder_add_block(gcb, 'BlockFactory', 'com.altera.dspbuilder.blockset.altlab.QuartusIIPinAssignment');  PostSaveFcn=alt_dspbuilder_block_saved(gcb);  NameChangeFcn=alt_dspbuilder_block_renamed(gcb);
      mask Help: helpview(char(com.altera.dspbuilder.simulation.Cache.getBlockTemplate('BlockFactory', 'com.altera.dspbuilder.blockset.altlab.QuartusIIPinAssignment').getHelpFile))
      mask Display:
      | plot([0 0 9 10 9 9 10 10 0],[0 10 10 7 7 10 7 0 0]);
      | fprintf('%s\n%s', QuartusIIAssignmentName, QuartusIIAssignmentValue);
  ROM : S-Function  LoadFcn=alt_dspbuilder_load_block(gcb, 'BlockFactory', 'com.altera.dspbuilder.blockset.storage.ROM');  FunctionName=sGeneric  Parameters=numwords BusType bwl bwr memory_type ram_type initialization init_file init_array register_outputs use_ena ClockPhase pipeline_display allowFloatingPointOverride logOutputs logFile enable_runtime_mod instance_name  EnableBusSupport=off  mask(ROM AlteraBlockset){numwords=16, BusType=Signed Integer, bwl=8, bwr=0, memory_type=AUTO, ram_type=ROM, initialization=From HEX file, init_file=input.hex, init_array=[0:1:15], register_outputs=off, use_ena=off, ClockPhase=1, pipeline_display=1, allowFloatingPointOverride=on, logOutputs=off, logFile=D:\\allblocks%5Falteradspbuilder2_ROM.fixedpointlog, enable_runtime_mod=off, instance_name=AAAA}
      mask prompts: numwords "Number Of Words (depth)"; BusType "Data Type"; bwl "[Number Of Bits].[]"; bwr "[].[Number Of Bits]"; memory_type "Memory Block Type"; ram_type "RAM type"; init_file "Input HEX File"; init_array "MATLAB Array"; register_outputs "Register Output Port"; use_ena "Use Enable Port (ena)"; ClockPhase "Clock Phase Selection"; pipeline_display "Number Of Pipeline Stages (Calculated)"; allowFloatingPointOverride "Allow Floating Point Override For This Block"; enable_runtime_mod "Create In-System Modifiable Memory"; instance_name "Instance ID (4 letters)"
      mask help:
      | Maps data to an embedded RAM in Altera devices, with read-only access.
      |
      | The ROM block can store any Data type. The address port is registered, and the data output port optionally registered.
      |
      | The contents of the ROM are pre-initialized from an Intel-format hexadecimal (.hex) file, or from a MATLAB array.
      |
      | You can use the Quartus II software to generate a .hex file. Any specified .hex file must be saved in your DSP Builder working directory.
      |
      | If used, the MATLAB array parameter must be a one dimensional MATLAB array with a length less than or equal to the number of words.
      | The array can be specified from the MATLAB work-space or directly in the MATLAB Array box.
      |
      | Note that the input address bus must be Unsigned, not all memory options are available for all device families, outputs must be registered for memory type MLAB and the clock enable (ena) bypasses any output register.
      mask init:
      | alt_dspbuilder_init('BlockFactory', 'com.altera.dspbuilder.blockset.storage.ROM', { numwords get_param(gcb, 'BusType') bwl bwr memory_type ram_type get_param(gcb, 'initialization') init_file init_array register_outputs get_param(gcb, 'use_ena') ClockPhase pipeline_display allowFloatingPointOverride logOutputs logFile get_param(gcb, 'enable_runtime_mod') instance_name });
      settings: CopyFcn=alt_dspbuilder_add_block(gcb, 'BlockFactory', 'com.altera.dspbuilder.blockset.storage.ROM');  DeleteFcn=com.altera.dspbuilder.simulation.Mask.delete(gcb);  UndoDeleteFcn=alt_dspbuilder_add_block(gcb, 'BlockFactory', 'com.altera.dspbuilder.blockset.storage.ROM');  PostSaveFcn=alt_dspbuilder_block_saved(gcb);  NameChangeFcn=alt_dspbuilder_block_renamed(gcb);
      mask Help: helpview(char(com.altera.dspbuilder.simulation.Cache.getBlockTemplate('BlockFactory', 'com.altera.dspbuilder.blockset.storage.ROM').getHelpFile))
      mask StyleString: edit,popup(Signed Integer|Unsigned Integer|Signed Fractional|Unsigned Fractional),edit,edit,popup(AUTO|M9K|M10K|M20K|MLAB|M144K),popup(ROM|SingleRAM|DualRAM|TrueDualRAM),popup(From HEX file|From MATLAB array),edit,edit,checkbox,checkbox,edit,edit,checkbox,checkbox,edit,checkbox,edit
      mask CallbackString: |alt_dspbuilder_update_gui('BlockFactory', 'com.altera.dspbuilder.blockset.storage.ROM', 'BusType', 1);|||||alt_dspbuilder_update_gui('BlockFactory', 'com.altera.dspbuilder.blockset.storage.ROM', 'initialization', 6);||||alt_dspbuilder_update_gui('BlockFactory', 'com.altera.dspbuilder.blockset.storage.ROM', 'use_ena', 10);||||||alt_dspbuilder_update_gui('BlockFactory', 'com.altera.dspbuilder.blockset.storage.ROM', 'enable_runtime_mod', 16);|
      mask TabNameString: Main,Main,Main,Main,Main,Main,Initialization,Initialization,Initialization,Registers and Enables,Registers and Enables,Registers and Enables,Registers and Enables,Registers and Enables,Registers and Enables,Registers and Enables,In-System Debug,In-System Debug
      mask Display:
      | port_label('input', 1, 'addr(3:0)');
      | port_label('output', 1, 'q(7:0)');
      | fprintf('ROM\n(%d x %d)' , 16, 8);
  Real-Imag to Complex : S-Function  LoadFcn=alt_dspbuilder_load_block(gcb, 'BlockFactory', 'com.altera.dspbuilder.blockset.complex.RealImagToComplex');  FunctionName=sGeneric  Parameters=BusType bwl bwr pipeline_display allowFloatingPointOverride logOutputs logFile  EnableBusSupport=off  mask(RealImagToComplex AlteraBlockset){BusType=Signed Integer, bwl=8, bwr=0, pipeline_display=0, allowFloatingPointOverride=on, logOutputs=off, logFile=D:\\allblocks%5Falteradspbuilder2_Real-Imag+to+Complex.fixedpointlog}
      mask prompts: BusType "Bus Type"; bwl "[Number Of Bits].[]"; bwr "[].[Number Of Bits]"; pipeline_display "Number Of Pipeline Stages (Calculated)"; allowFloatingPointOverride "Allow Floating Point Override For This Block"
      mask help: Constructs a fixed-point complex output from a fixed-point real input and a fixed-point imaginary input.
      mask init:
      | alt_dspbuilder_init('BlockFactory', 'com.altera.dspbuilder.blockset.complex.RealImagToComplex', { get_param(gcb, 'BusType') bwl bwr pipeline_display allowFloatingPointOverride logOutputs logFile });
      settings: CopyFcn=alt_dspbuilder_add_block(gcb, 'BlockFactory', 'com.altera.dspbuilder.blockset.complex.RealImagToComplex');  DeleteFcn=com.altera.dspbuilder.simulation.Mask.delete(gcb);  UndoDeleteFcn=alt_dspbuilder_add_block(gcb, 'BlockFactory', 'com.altera.dspbuilder.blockset.complex.RealImagToComplex');  PostSaveFcn=alt_dspbuilder_block_saved(gcb);  NameChangeFcn=alt_dspbuilder_block_renamed(gcb);
      mask Help: helpview(char(com.altera.dspbuilder.simulation.Cache.getBlockTemplate('BlockFactory', 'com.altera.dspbuilder.blockset.complex.RealImagToComplex').getHelpFile))
      mask StyleString: popup(Signed Integer|Unsigned Integer|Signed Fractional|Unsigned Fractional),edit,edit,edit,checkbox,checkbox,edit
      mask CallbackString: alt_dspbuilder_update_gui('BlockFactory', 'com.altera.dspbuilder.blockset.complex.RealImagToComplex', 'BusType', 0);||||||
      mask Display:
      | port_label('input', 1, 'r (7:0)');
      | port_label('input', 2, 'i (7:0)');
      | port_label('output', 1, 'c (7:0)');
  Resource Usage : S-Function  LoadFcn=alt_dspbuilder_load_block(gcb, 'BlockFactory', 'com.altera.dspbuilder.blockset.altlab.ResourceUsage');  FunctionName=sNoOp  Parameters=logic memory dsp memoryLable dspLable  EnableBusSupport=off  mask(Resource Usage AlteraBlockset){logic=N/A, memory=N/A, dsp=N/A, memoryLable=RAM, dspLable=DSP}
      mask prompts: memoryLable "Memory Lable"; dspLable "DSP Lable"
      mask init:
      | alt_dspbuilder_init('BlockFactory', 'com.altera.dspbuilder.blockset.altlab.ResourceUsage', { logic memory dsp memoryLable dspLable });
      settings: CopyFcn=alt_dspbuilder_add_block(gcb, 'BlockFactory', 'com.altera.dspbuilder.blockset.altlab.ResourceUsage');  DeleteFcn=com.altera.dspbuilder.simulation.Mask.delete(gcb);  UndoDeleteFcn=alt_dspbuilder_add_block(gcb, 'BlockFactory', 'com.altera.dspbuilder.blockset.altlab.ResourceUsage');  PostSaveFcn=alt_dspbuilder_block_saved(gcb);  NameChangeFcn=alt_dspbuilder_block_renamed(gcb);
      settings: OpenFcn=|
      | com.altera.dspbuilder.simulation.Mask.simpleInit('BlockFactory', 'com.altera.dspbuilder.blockset.altlab.ResourceUsage', bdroot(gcb), gcb);
      | alt_dspbuilder_resourceusageLaunch(gcb)
      mask Help: helpview(char(com.altera.dspbuilder.simulation.Cache.getBlockTemplate('BlockFactory', 'com.altera.dspbuilder.blockset.altlab.ResourceUsage').getHelpFile))
      mask Display: fprintf('Logic: N/A\nRAM: N/A\nDSP: N/A');
  Round : S-Function  LoadFcn=alt_dspbuilder_load_block(gcb, 'BlockFactory', 'com.altera.dspbuilder.blockset.iobus.Round');  FunctionName=sGeneric  Parameters=BusType bwl bwr bitsToRemove roundMode userRoundMode pipeline pipeline_display use_ena use_aclr  EnableBusSupport=off  mask(Round AlteraBlockset){BusType=Signed Integer, bwl=8, bwr=1, bitsToRemove=0, roundMode=TRUNCATE_LOW, userRoundMode=Truncate, pipeline=off, pipeline_display=0, use_ena=off, use_aclr=off}
      mask prompts: BusType "Bus Type"; bwl "[Number Of Bits].[]"; bwr "[].[Number Of Bits]"; bitsToRemove "Number Of LSB Bits To Remove"; userRoundMode "Rounding Mode"; pipeline "Enable Pipeline"; pipeline_display "Number Of Pipeline Stages (Calculated)"; use_ena "Use Enable Port (ena)"; use_aclr "Use Asynchronous Clear Port (aclr)"
      mask help:
      | Rounds the input to the closest possible representation in the specified output bus format.
      |
      | If the nearest two possibilities are equidistant, you can choose from the available rounding modes:
      | Truncate - Remove discarded bits without changing the other bits (effectively, choose the lower value).
      | Round Towards Zero - Choose the value closer to zero.
      | Round Away From Zero - Choose the value further from zero (i.e. round downwards for negative values, upwards for positive values).
      | Round To Plus Infinity - Choose the higher value.
      | Convergent Rounding - Choose the even value.
      |
      | For more information on rounding modes, see the help file for this block.
      mask init:
      | alt_dspbuilder_init('BlockFactory', 'com.altera.dspbuilder.blockset.iobus.Round', { get_param(gcb, 'BusType') bwl bwr bitsToRemove roundMode userRoundMode get_param(gcb, 'pipeline') pipeline_display get_param(gcb, 'use_ena') get_param(gcb, 'use_aclr') });
      settings: CopyFcn=alt_dspbuilder_add_block(gcb, 'BlockFactory', 'com.altera.dspbuilder.blockset.iobus.Round');  DeleteFcn=com.altera.dspbuilder.simulation.Mask.delete(gcb);  UndoDeleteFcn=alt_dspbuilder_add_block(gcb, 'BlockFactory', 'com.altera.dspbuilder.blockset.iobus.Round');  PostSaveFcn=alt_dspbuilder_block_saved(gcb);  NameChangeFcn=alt_dspbuilder_block_renamed(gcb);
      mask Help: helpview(char(com.altera.dspbuilder.simulation.Cache.getBlockTemplate('BlockFactory', 'com.altera.dspbuilder.blockset.iobus.Round').getHelpFile))
      mask StyleString: popup(Signed Integer|Unsigned Integer|Signed Fractional|Unsigned Fractional),edit,edit,edit,edit,popup(Truncate|Round Towards Zero|Round Away From Zero|Round To Plus Infinity|Convergent Rounding),checkbox,edit,checkbox,checkbox
      mask CallbackString: alt_dspbuilder_update_gui('BlockFactory', 'com.altera.dspbuilder.blockset.iobus.Round', 'BusType', 0);||||||alt_dspbuilder_update_gui('BlockFactory', 'com.altera.dspbuilder.blockset.iobus.Round', 'pipeline', 6);||alt_dspbuilder_update_gui('BlockFactory', 'com.altera.dspbuilder.blockset.iobus.Round', 'use_ena', 8);|alt_dspbuilder_update_gui('BlockFactory', 'com.altera.dspbuilder.blockset.iobus.Round', 'use_aclr', 9);
      mask TabNameString: Main,Main,Main,Main,Main,Main,Main,Main,Optional Ports,Optional Ports
      mask Display:
      | port_label('input', 1, '(7:0)');
      | port_label('output', 1, '(7:0)');
      | plot([0.5 0.5 0 0 1], [1 0 0 1 1])
  SOP Tap : S-Function  LoadFcn=alt_dspbuilder_load_block(gcb, 'BlockFactory', 'com.altera.dspbuilder.blockset.arithmetic.SOPTAP');  FunctionName=sGeneric  Parameters=BusType bwl bwr number_of_taps pipeline_display use_ena use_aclr allowFloatingPointOverride logOutputs logFile  EnableBusSupport=off  mask(SOP Tap AlteraBlockset){BusType=Signed Integer, bwl=8, bwr=0, number_of_taps=2, pipeline_display=2, use_ena=off, use_aclr=off, allowFloatingPointOverride=on, logOutputs=off, logFile=D:\\allblocks%5Falteradspbuilder2_SOP+Tap%3A%3Aq.fixedpointlog,D:\\allblocks%5Falteradspbuilder2_SOP+Tap%3A%3Adout.fixedpointlog,}
      mask prompts: BusType "Bus Type"; bwl "[Number Of Bits].[]"; bwr "[].[Number Of Bits]"; number_of_taps "Number Of Taps (2 or 4)"; pipeline_display "Number Of Pipeline Stages (Calculated)"; use_ena "Use Enable Port (ena)"; use_aclr "Use Asynchronous Clear Port (aclr)"; allowFloatingPointOverride "Allow Floating Point Override For This Block"
      mask help:
      | Performs a sum of products for two or four taps. You can use this block to build two or four tap FIR filters, or cascade blocks to create filters with more taps.
      |
      | The SOP Tap block is implemented using a multiplier-adder which has registers on the inputs, multipliers and adders. Thus, the result always lags the input by 3 cycles. The dout port is assigned the value of din(n-t) where t is the number of taps. The block has the equations:
      |
      | For 2 taps:
      |   q(n+3) = c0(n) x din(n) + c1(n) x din(n-1)
      |   dout(n+2) = din(n)
      |
      | For 4 taps:
      |   q(n+3) = c0(n) x din(n) + c1(n) x din(n-1) + c2(n) x din(n-2) + c3(n) x din(n-3)
      |   dout(n+4) = din(n)
      mask init:
      | alt_dspbuilder_init('BlockFactory', 'com.altera.dspbuilder.blockset.arithmetic.SOPTAP', { get_param(gcb, 'BusType') bwl bwr number_of_taps pipeline_display use_ena use_aclr allowFloatingPointOverride logOutputs logFile });
      settings: CopyFcn=alt_dspbuilder_add_block(gcb, 'BlockFactory', 'com.altera.dspbuilder.blockset.arithmetic.SOPTAP');  DeleteFcn=com.altera.dspbuilder.simulation.Mask.delete(gcb);  UndoDeleteFcn=alt_dspbuilder_add_block(gcb, 'BlockFactory', 'com.altera.dspbuilder.blockset.arithmetic.SOPTAP');  PostSaveFcn=alt_dspbuilder_block_saved(gcb);  NameChangeFcn=alt_dspbuilder_block_renamed(gcb);
      mask Help: helpview(char(com.altera.dspbuilder.simulation.Cache.getBlockTemplate('BlockFactory', 'com.altera.dspbuilder.blockset.arithmetic.SOPTAP').getHelpFile))
      mask StyleString: popup(Signed Integer|Unsigned Integer|Signed Fractional|Unsigned Fractional),edit,edit,popup(2|4),edit,checkbox,checkbox,checkbox,checkbox,edit
      mask CallbackString: alt_dspbuilder_update_gui('BlockFactory', 'com.altera.dspbuilder.blockset.arithmetic.SOPTAP', 'BusType', 0);|||||||||
      mask TabNameString: Main,Main,Main,Main,Main,Optional Ports,Optional Ports,Optional Ports,Optional Ports,Optional Ports
      mask Display:
      | port_label('input', 1, 'din(7:0)');
      | port_label('input', 2, 'c0(7:0)');
      | port_label('input', 3, 'c1(7:0)');
      | port_label('output', 1, 'q(16:0)');
      | port_label('output', 2, 'dout(7:0)');
      | disp('SOP');
  Saturate : S-Function  LoadFcn=alt_dspbuilder_load_block(gcb, 'BlockFactory', 'com.altera.dspbuilder.blockset.iobus.Saturate');  FunctionName=sGeneric  Parameters=BusType bwl bwr bitsToRemove satMode UpperLimit LowerLimit pipeline pipeline_display use_sat_flag use_ena use_aclr  EnableBusSupport=off  mask(Saturate AlteraBlockset){BusType=Signed Integer, bwl=8, bwr=0, bitsToRemove=0, satMode=Truncate MSB, UpperLimit=0, LowerLimit=0, pipeline=off, pipeline_display=0, use_sat_flag=off, use_ena=off, use_aclr=off}
      mask prompts: BusType "Bus Type"; bwl "[Number Of Bits].[]"; bwr "[].[Number Of Bits]"; bitsToRemove "Number Of MSB Bits To Remove"; satMode "Saturation Type"; UpperLimit "Upper Saturation Limit"; LowerLimit "Lower Saturation Limit"; pipeline "Enable Pipeline"; pipeline_display "Number Of Pipeline Stages (Calculated)"; use_sat_flag "Use optional saturation occurred port"; use_ena "Use Enable Port (ena)"; use_aclr "Use Asynchronous Clear Port (aclr)"
      mask help: Limits output to a maximum value. If the output is greater than the maximum positive or negative value to be represented, the output is forced (or saturated) to the maximum positive or negative value, respectively. Alternatively, you can choose to truncate the MSB.
      mask init:
      | alt_dspbuilder_init('BlockFactory', 'com.altera.dspbuilder.blockset.iobus.Saturate', { get_param(gcb, 'BusType') bwl bwr bitsToRemove get_param(gcb, 'satMode') UpperLimit LowerLimit get_param(gcb, 'pipeline') pipeline_display get_param(gcb, 'use_sat_flag') get_param(gcb, 'use_ena') get_param(gcb, 'use_aclr') });
      settings: CopyFcn=alt_dspbuilder_add_block(gcb, 'BlockFactory', 'com.altera.dspbuilder.blockset.iobus.Saturate');  DeleteFcn=com.altera.dspbuilder.simulation.Mask.delete(gcb);  UndoDeleteFcn=alt_dspbuilder_add_block(gcb, 'BlockFactory', 'com.altera.dspbuilder.blockset.iobus.Saturate');  PostSaveFcn=alt_dspbuilder_block_saved(gcb);  NameChangeFcn=alt_dspbuilder_block_renamed(gcb);
      mask Help: helpview(char(com.altera.dspbuilder.simulation.Cache.getBlockTemplate('BlockFactory', 'com.altera.dspbuilder.blockset.iobus.Saturate').getHelpFile))
      mask StyleString: popup(Signed Integer|Unsigned Integer|Signed Fractional|Unsigned Fractional),edit,edit,edit,popup(Saturate|Truncate MSB|Enter Saturation Limits),edit,edit,checkbox,edit,checkbox,checkbox,checkbox
      mask CallbackString: alt_dspbuilder_update_gui('BlockFactory', 'com.altera.dspbuilder.blockset.iobus.Saturate', 'BusType', 0);||||alt_dspbuilder_update_gui('BlockFactory', 'com.altera.dspbuilder.blockset.iobus.Saturate', 'satMode', 4);|||alt_dspbuilder_update_gui('BlockFactory', 'com.altera.dspbuilder.blockset.iobus.Saturate', 'pipeline', 7);||alt_dspbuilder_update_gui('BlockFactory', 'com.altera.dspbuilder.blockset.iobus.Saturate', 'use_sat_flag', 9);|alt_dspbuilder_update_gui('BlockFactory', 'com.altera.dspbuilder.blockset.iobus.Saturate', 'use_ena', 10);|alt_dspbuilder_update_gui('BlockFactory', 'com.altera.dspbuilder.blockset.iobus.Saturate', 'use_aclr', 11);
      mask TabNameString: Main,Main,Main,Main,Main,Main,Main,Main,Main,Optional Ports,Optional Ports,Optional Ports
      mask Display:
      | port_label('input', 1, '(7:0)');
      | port_label('output', 1, '(7:0)');
      | plot([0.5 0.5 0 0 1], [1 0 0 1 1])
  Serial To Parallel : S-Function  LoadFcn=alt_dspbuilder_load_block(gcb, 'BlockFactory', 'com.altera.dspbuilder.blockset.storage.SerialToParallel');  FunctionName=sGeneric  Parameters=BusType bwl bwr msbfirsttext msbfirst use_ena use_sclr  EnableBusSupport=off  mask(Serial To Parallel AlteraBlockset){BusType=Signed Integer, bwl=8, bwr=0, msbfirsttext=MSB First, msbfirst=1, use_ena=on, use_sclr=on}
      mask prompts: BusType "Data Bus Type"; bwl "[Number Of Bits].[]"; bwr "[].[Number Of Bits]"; msbfirsttext "Serial Bit Order"; msbfirst "Serial Bit Order Boolean"; use_ena "Use Enable Port (ena)"; use_sclr "Use Synchronous Clear port (sclr)"
      mask help:
      | Implements a serial (input sd) to parallel bus conversion (output d).
      |
      | The input bit stream can be treated as either most significant bit (MSB) first, or least significant bit (LSB) first.
      mask init:
      | alt_dspbuilder_init('BlockFactory', 'com.altera.dspbuilder.blockset.storage.SerialToParallel', { get_param(gcb, 'BusType') bwl bwr msbfirsttext msbfirst use_ena use_sclr });
      settings: CopyFcn=alt_dspbuilder_add_block(gcb, 'BlockFactory', 'com.altera.dspbuilder.blockset.storage.SerialToParallel');  DeleteFcn=com.altera.dspbuilder.simulation.Mask.delete(gcb);  UndoDeleteFcn=alt_dspbuilder_add_block(gcb, 'BlockFactory', 'com.altera.dspbuilder.blockset.storage.SerialToParallel');  PostSaveFcn=alt_dspbuilder_block_saved(gcb);  NameChangeFcn=alt_dspbuilder_block_renamed(gcb);
      mask Help: helpview(char(com.altera.dspbuilder.simulation.Cache.getBlockTemplate('BlockFactory', 'com.altera.dspbuilder.blockset.storage.SerialToParallel').getHelpFile))
      mask StyleString: popup(Signed Integer|Unsigned Integer|Signed Fractional|Unsigned Fractional),edit,edit,popup(MSB First|LSB First),edit,checkbox,checkbox
      mask CallbackString: alt_dspbuilder_update_gui('BlockFactory', 'com.altera.dspbuilder.blockset.storage.SerialToParallel', 'BusType', 0);||||||
      mask TabNameString: Main,Main,Main,Main,Main,Optional Ports,Optional Ports
      mask Display:
      | port_label('input', 1, 'sd');
      | port_label('input', 2, 'ena');
      | port_label('input', 3, 'sclr');
      | port_label('output', 1, 'd(7:0)');
  Shift Taps : S-Function  LoadFcn=alt_dspbuilder_load_block(gcb, 'BlockFactory', 'com.altera.dspbuilder.blockset.storage.ShiftTaps');  FunctionName=sGeneric  Parameters=number_of_taps tap_distance use_shiftout use_ena use_sclr use_dedicated_circuitry ram_type allowFloatingPointOverride logOutputs logFile  EnableBusSupport=off  mask(Shift Taps AlteraBlockset){number_of_taps=1, tap_distance=1, use_shiftout=off, use_ena=off, use_sclr=off, use_dedicated_circuitry=off, ram_type=AUTO, allowFloatingPointOverride=on, logOutputs=off, logFile=D:\\allblocks%5Falteradspbuilder2_Shift+Taps.fixedpointlog}
      mask prompts: number_of_taps "Number Of Taps"; tap_distance "Distance Between Taps"; use_shiftout "Use Shift Out Port"; use_ena "Use Enable Port (ena)"; use_sclr "Use Synchronous Clear Port (sclr)"; use_dedicated_circuitry "Use Dedicated Circuitry (if tap distance > 2)"; ram_type "Memory Block Type"; allowFloatingPointOverride "Allow Floating Point Override For This Block"
      mask help:
      | Implements a shift register that you can use for filters or convolution.
      |
      | The 'Use Dedicated Circuitry' option uses the device's embedded memory blocks, when possible. This option is only available when the 'Distance between taps' is greater than 2.
      |
      | Note; not all memory options are available for all device families.
      mask init:
      | alt_dspbuilder_init('BlockFactory', 'com.altera.dspbuilder.blockset.storage.ShiftTaps', { number_of_taps tap_distance use_shiftout use_ena use_sclr get_param(gcb, 'use_dedicated_circuitry') ram_type allowFloatingPointOverride logOutputs logFile });
      settings: CopyFcn=alt_dspbuilder_add_block(gcb, 'BlockFactory', 'com.altera.dspbuilder.blockset.storage.ShiftTaps');  DeleteFcn=com.altera.dspbuilder.simulation.Mask.delete(gcb);  UndoDeleteFcn=alt_dspbuilder_add_block(gcb, 'BlockFactory', 'com.altera.dspbuilder.blockset.storage.ShiftTaps');  PostSaveFcn=alt_dspbuilder_block_saved(gcb);  NameChangeFcn=alt_dspbuilder_block_renamed(gcb);
      mask Help: helpview(char(com.altera.dspbuilder.simulation.Cache.getBlockTemplate('BlockFactory', 'com.altera.dspbuilder.blockset.storage.ShiftTaps').getHelpFile))
      mask StyleString: edit,edit,checkbox,checkbox,checkbox,checkbox,popup(AUTO|M9K|M10K|M20K|MLAB|M144K),checkbox,checkbox,edit
      mask CallbackString: |||||alt_dspbuilder_update_gui('BlockFactory', 'com.altera.dspbuilder.blockset.storage.ShiftTaps', 'use_dedicated_circuitry', 5);||||
      mask TabNameString: Main,Main,Optional Ports and Settings,Optional Ports and Settings,Optional Ports and Settings,Optional Ports and Settings,Optional Ports and Settings,Optional Ports and Settings,Optional Ports and Settings,Optional Ports and Settings
      mask Display:
      | port_label('input', 1, 'd');
      | port_label('output', 1, 't0');
      | 
      | disp('1 tap','texmode','on');
  Signal Compiler : S-Function  LoadFcn=alt_dspbuilder_load_block(gcb, 'BlockFactory', 'com.altera.dspbuilder.blockset.altlab.SignalCompiler');  FunctionName=sNoOp  EnableBusSupport=off  mask(Signal Compiler AlteraBlockset){DeviceFamily=Stratix III, DeviceName=AUTO, DisableEarlyHDLGeneration=off, EnableSignalTap=off, SignalTapDepth=128, UseBoardBlock=off, StpUseDefaultClock=on, StpClock=clock, ExportDir=.}
      mask prompts: DeviceFamily "Device Family"; DeviceName "Device Name"; DisableEarlyHDLGeneration "Disable Early HDL Generation"; EnableSignalTap "Enable SignalTap"; SignalTapDepth "SignalTap Depth"; UseBoardBlock "Use Board Block"; StpUseDefaultClock "Use Default Clock for SignalTap II"; StpClock "SignalTap II Clock"; ExportDir "Export Directory"
      mask help:
      | Controls the compilation of the design in the Quartus II software.
      |
      | Your model file must be saved before you can use the Signal Compiler block.
      mask init:
      | alt_dspbuilder_init_signalcompiler('BlockFactory', 'com.altera.dspbuilder.blockset.altlab.SignalCompiler', { DeviceFamily DeviceName DisableEarlyHDLGeneration EnableSignalTap SignalTapDepth UseBoardBlock StpUseDefaultClock StpClock ExportDir });
      settings: CopyFcn=alt_dspbuilder_add_block(gcb, 'BlockFactory', 'com.altera.dspbuilder.blockset.altlab.SignalCompiler');  DeleteFcn=com.altera.dspbuilder.simulation.Mask.delete(gcb);  UndoDeleteFcn=alt_dspbuilder_add_block(gcb, 'BlockFactory', 'com.altera.dspbuilder.blockset.altlab.SignalCompiler');  PostSaveFcn=alt_dspbuilder_block_saved(gcb);  NameChangeFcn=alt_dspbuilder_block_renamed(gcb);
      settings: OpenFcn=|
      | com.altera.dspbuilder.simulation.Mask.simpleInit('BlockFactory', 'com.altera.dspbuilder.blockset.altlab.SignalCompiler', bdroot(gcb), gcb);
      | alt_signalcompilerLaunch(gcb)
      mask Help: helpview(char(com.altera.dspbuilder.simulation.Cache.getBlockTemplate('BlockFactory', 'com.altera.dspbuilder.blockset.altlab.SignalCompiler').getHelpFile))
      mask Display: image(imread('SIGCOMP64X64.bmp', 'bmp'));
  SignalTap II Logic Analyzer : S-Function  LoadFcn=alt_dspbuilder_load_block(gcb, 'BlockFactory', 'com.altera.dspbuilder.blockset.altlab.SignalTapAnalyzer');  FunctionName=sNoOp  EnableBusSupport=off  mask(SignalTap Analyzer AlteraBlockset){}
      mask help: Configures the SignalTap II embedded logic analyzer and retrieves tapped data.
      mask init:
      | alt_dspbuilder_init('BlockFactory', 'com.altera.dspbuilder.blockset.altlab.SignalTapAnalyzer', { });
      settings: CopyFcn=alt_dspbuilder_add_block(gcb, 'BlockFactory', 'com.altera.dspbuilder.blockset.altlab.SignalTapAnalyzer');  DeleteFcn=com.altera.dspbuilder.simulation.Mask.delete(gcb);  UndoDeleteFcn=alt_dspbuilder_add_block(gcb, 'BlockFactory', 'com.altera.dspbuilder.blockset.altlab.SignalTapAnalyzer');  PostSaveFcn=alt_dspbuilder_block_saved(gcb);  NameChangeFcn=alt_dspbuilder_block_renamed(gcb);
      settings: OpenFcn=|
      | com.altera.dspbuilder.simulation.Mask.simpleInit('BlockFactory', 'com.altera.dspbuilder.blockset.altlab.SignalTapAnalyzer', bdroot(gcb), gcb);
      | alt_signaltapLaunch(gcb)
      mask Help: helpview(char(com.altera.dspbuilder.simulation.Cache.getBlockTemplate('BlockFactory', 'com.altera.dspbuilder.blockset.altlab.SignalTapAnalyzer').getHelpFile))
      mask Display: image(imread('SSIGNALTAP.bmp', 'bmp'));
  SignalTap II Node : S-Function  LoadFcn=alt_dspbuilder_load_block(gcb, 'BlockFactory', 'com.altera.dspbuilder.blockset.altlab.SignalTapNode');  FunctionName=sGeneric  Parameters=id  EnableBusSupport=off  mask(SignalTap Node AlteraBlockset){id=0}
      mask prompts: id "unique id"
      mask help: Used with the SignalTap II Logic Analyzer block to capture signal activity from your design as it runs in hardware.
      mask init:
      | alt_dspbuilder_init('BlockFactory', 'com.altera.dspbuilder.blockset.altlab.SignalTapNode', { id });
      settings: DeleteFcn=com.altera.dspbuilder.simulation.Mask.delete(gcb);  UndoDeleteFcn=alt_dspbuilder_add_block(gcb, 'BlockFactory', 'com.altera.dspbuilder.blockset.altlab.SignalTapNode');  PostSaveFcn=alt_dspbuilder_block_saved(gcb);  NameChangeFcn=alt_dspbuilder_block_renamed(gcb);
      settings: CopyFcn=|
      | alt_dspbuilder_add_block(gcb, 'BlockFactory', 'com.altera.dspbuilder.blockset.altlab.SignalTapNode');
      | com.altera.dspbuilder.simulation.Mask.simpleInit('BlockFactory', 'com.altera.dspbuilder.blockset.altlab.SignalTapNode', bdroot(gcb), gcb);
      | alt_dspbuilder_internal_init_uniqueidblock(gcb);
      mask Help: helpview(char(com.altera.dspbuilder.simulation.Cache.getBlockTemplate('BlockFactory', 'com.altera.dspbuilder.blockset.altlab.SignalTapNode').getHelpFile))
      mask Display:
      | disp('SignalTap II');
      | plot([0 1 2 1 0],[0 2 0 -2 0]);
  Single Pulse : S-Function  LoadFcn=alt_dspbuilder_load_block(gcb, 'BlockFactory', 'com.altera.dspbuilder.blockset.gatecontrol.SinglePulse');  FunctionName=sGeneric  Parameters=signal_type impulse_width delay SpecifyClock use_ena use_sclr  EnableBusSupport=off  mask(Single Pulse AlteraBlockset){signal_type=Step Up, impulse_width=1, delay=1, SpecifyClock=off, clock=, use_ena=off, use_sclr=off}
      mask prompts: signal_type "Signal Generation Type"; impulse_width "Impulse Length"; SpecifyClock "Specify Clock"; use_ena "Use Enable Port (ena)"; use_sclr "Use Synchronous Clear Port (sclr)"
      mask help:
      | Generates a single pulse output signal. The output signal is a single bit that takes only the values 1 or 0. The signal generation type could be an Impulse, a Step Up (0 to 1), or a Step Down (1 to 0)
      |
      | The output of a Impulse starts at 0 changing to 1 after a specified delay and changing to 0 again after a specified length. The output of a Step Up starts at 0 changing to 1 after a specified delay. The output of a Step Down starts at 1 changing to 0 after a specified delay.
      |
      | Note: This block is synchronously reset, however on the next cycle the block will be active, that is it takes 0 cycles to reset.
      mask init:
      | alt_dspbuilder_init('BlockFactory', 'com.altera.dspbuilder.blockset.gatecontrol.SinglePulse', { get_param(gcb, 'signal_type') impulse_width delay get_param(gcb, 'SpecifyClock') clock use_ena use_sclr });
      settings: CopyFcn=alt_dspbuilder_add_block(gcb, 'BlockFactory', 'com.altera.dspbuilder.blockset.gatecontrol.SinglePulse');  DeleteFcn=com.altera.dspbuilder.simulation.Mask.delete(gcb);  UndoDeleteFcn=alt_dspbuilder_add_block(gcb, 'BlockFactory', 'com.altera.dspbuilder.blockset.gatecontrol.SinglePulse');  PostSaveFcn=alt_dspbuilder_block_saved(gcb);  NameChangeFcn=alt_dspbuilder_block_renamed(gcb);
      mask Help: helpview(char(com.altera.dspbuilder.simulation.Cache.getBlockTemplate('BlockFactory', 'com.altera.dspbuilder.blockset.gatecontrol.SinglePulse').getHelpFile))
      mask StyleString: popup(Step Up|Step Down|Impulse),edit,edit,checkbox,edit,checkbox,checkbox
      mask CallbackString: alt_dspbuilder_update_gui('BlockFactory', 'com.altera.dspbuilder.blockset.gatecontrol.SinglePulse', 'signal_type', 0);|||alt_dspbuilder_update_gui('BlockFactory', 'com.altera.dspbuilder.blockset.gatecontrol.SinglePulse', 'SpecifyClock', 3);|||
      mask TabNameString: Main,Main,Main,Main,Main,Optional Ports,Optional Ports
      mask Display: plot([0 45 45 70], [0 0 60 60]);
  Single-Port RAM : S-Function  LoadFcn=alt_dspbuilder_load_block(gcb, 'BlockFactory', 'com.altera.dspbuilder.blockset.storage.SingleRam');  FunctionName=sGeneric  Parameters=numwords BusType bwl bwr memory_type ram_type initialization init_file init_array register_outputs use_ena ClockPhase pipeline_display allowFloatingPointOverride logOutputs logFile enable_runtime_mod instance_name  EnableBusSupport=off  mask(Single-Port RAM AlteraBlockset){numwords=16, BusType=Signed Integer, bwl=8, bwr=0, memory_type=AUTO, ram_type=SingleRAM, initialization=Blank, init_file=input.hex, init_array=[0:1:15], register_outputs=off, use_ena=off, ClockPhase=1, pipeline_display=1, allowFloatingPointOverride=on, logOutputs=off, logFile=D:\\allblocks%5Falteradspbuilder2_Single-Port+RAM.fixedpointlog, enable_runtime_mod=off, instance_name=AAAA}
      mask prompts: numwords "Number Of Words"; BusType "Data Type"; bwl "[Number Of Bits].[]"; bwr "[].[Number Of Bits]"; memory_type "Memory Block Type"; ram_type "RAM type"; init_file "Input HEX File"; init_array "MATLAB Array"; register_outputs "Register Output Port"; use_ena "Use Enable Port (ena)"; ClockPhase "Clock Phase Selection"; pipeline_display "Number Of Pipeline Stages (Calculated)"; allowFloatingPointOverride "Allow Floating Point Override For This Block"; enable_runtime_mod "Create In-System Modifiable Memory"; instance_name "Instance ID (4 letters)"
      mask help:
      | Maps data to an embedded RAM in Altera devices. A single read/write port allow simple access.
      |
      | The Single-Port RAM block accepts any type as Data input. The input port is registered, and the output port optionally registered.
      |
      | By default the contents of the RAM are pre-initialized to zero, but can be specified from an Intel-format hexadecimal (.hex) file, or from a MATLAB array.
      |
      | You can use the Quartus II software to generate a .hex file. Any specified .hex file must be saved in your DSP Builder working directory.
      |
      | If used, the MATLAB array parameter must be a one dimensional MATLAB array with a length less than or equal to the number of words.
      | The array can be specified from the MATLAB work-space or directly in the MATLAB Array box.
      |
      | Note that the input address bus must be Unsigned, not all memory options are available for all device families, initialization is not possible for memory type M-RAM, outputs must be registered for memory type MLAB, and the clock enable (ena) bypasses any output register.
      mask init:
      | alt_dspbuilder_init('BlockFactory', 'com.altera.dspbuilder.blockset.storage.SingleRam', { numwords get_param(gcb, 'BusType') bwl bwr get_param(gcb, 'memory_type') ram_type get_param(gcb, 'initialization') init_file init_array register_outputs get_param(gcb, 'use_ena') ClockPhase pipeline_display allowFloatingPointOverride logOutputs logFile get_param(gcb, 'enable_runtime_mod') instance_name });
      settings: CopyFcn=alt_dspbuilder_add_block(gcb, 'BlockFactory', 'com.altera.dspbuilder.blockset.storage.SingleRam');  DeleteFcn=com.altera.dspbuilder.simulation.Mask.delete(gcb);  UndoDeleteFcn=alt_dspbuilder_add_block(gcb, 'BlockFactory', 'com.altera.dspbuilder.blockset.storage.SingleRam');  PostSaveFcn=alt_dspbuilder_block_saved(gcb);  NameChangeFcn=alt_dspbuilder_block_renamed(gcb);
      mask Help: helpview(char(com.altera.dspbuilder.simulation.Cache.getBlockTemplate('BlockFactory', 'com.altera.dspbuilder.blockset.storage.SingleRam').getHelpFile))
      mask StyleString: edit,popup(Inferred|Signed Integer|Unsigned Integer|Signed Fractional|Unsigned Fractional),edit,edit,popup(AUTO|M9K|M10K|M20K|MLAB|M144K),popup(ROM|SingleRAM|DualRAM|TrueDualRAM),popup(Blank|From HEX file|From MATLAB array),edit,edit,checkbox,checkbox,edit,edit,checkbox,checkbox,edit,checkbox,edit
      mask CallbackString: |alt_dspbuilder_update_gui('BlockFactory', 'com.altera.dspbuilder.blockset.storage.SingleRam', 'BusType', 1);|||alt_dspbuilder_update_gui('BlockFactory', 'com.altera.dspbuilder.blockset.storage.SingleRam', 'memory_type', 4);||alt_dspbuilder_update_gui('BlockFactory', 'com.altera.dspbuilder.blockset.storage.SingleRam', 'initialization', 6);||||alt_dspbuilder_update_gui('BlockFactory', 'com.altera.dspbuilder.blockset.storage.SingleRam', 'use_ena', 10);||||||alt_dspbuilder_update_gui('BlockFactory', 'com.altera.dspbuilder.blockset.storage.SingleRam', 'enable_runtime_mod', 16);|
      mask TabNameString: Main,Main,Main,Main,Main,Main,Initialization,Initialization,Initialization,Registers and Enables,Registers and Enables,Registers and Enables,Registers and Enables,Registers and Enables,Registers and Enables,Registers and Enables,In-System Debug,In-System Debug
      mask Display:
      | port_label('input', 1, 'd(7:0)');
      | port_label('input', 2, 'addr(3:0)');
      | port_label('input', 3, 'wren');
      | port_label('output', 1, 'q');
      | fprintf('RAM\n(%d x %d)' , 16, 8);
  Square Root : S-Function  LoadFcn=alt_dspbuilder_load_block(gcb, 'BlockFactory', 'com.altera.dspbuilder.blockset.arithmetic.SquareRoot');  FunctionName=sGeneric  Parameters=BusType bwl bwr pipeline pipeline_display use_remain use_ena use_aclr  EnableBusSupport=off  mask(Square Root AlteraBlockset){BusType=Unsigned Integer, bwl=8, bwr=0, pipeline=0, pipeline_display=0, use_remain=off, use_ena=off, use_aclr=off}
      mask prompts: BusType "Bus Type"; bwl "Input Number of Bits"; bwr "Bit Width Right"; pipeline "Number of Pipeline Stages"; pipeline_display "Number Of Pipeline Stages (Calculated)"; use_remain "Use Remainder Port (remainder)"; use_ena "Use Enable Port (ena)"; use_aclr "Use Asynchronous Clear Port (aclr)"
      mask help:
      | Returns the square root and optional remainder of unsigned integer input data using the equation:
      |   q^2 + remainder = d
      |   where remainder <= 2 x q
      |
      | The Square Root block supports sequential mode (when the number of pipeline stages> 0) or combinational mode (when the number of pipeline stages = 0).
      |
      | Note that the radical, d, is assumed to be unsigned integer, and that q and the remainder are always unsigned integer.
      |
      | The expected results are the square root of the radical and the remainder.
      mask init:
      | alt_dspbuilder_init('BlockFactory', 'com.altera.dspbuilder.blockset.arithmetic.SquareRoot', { BusType bwl bwr pipeline pipeline_display get_param(gcb, 'use_remain') use_ena use_aclr });
      settings: CopyFcn=alt_dspbuilder_add_block(gcb, 'BlockFactory', 'com.altera.dspbuilder.blockset.arithmetic.SquareRoot');  DeleteFcn=com.altera.dspbuilder.simulation.Mask.delete(gcb);  UndoDeleteFcn=alt_dspbuilder_add_block(gcb, 'BlockFactory', 'com.altera.dspbuilder.blockset.arithmetic.SquareRoot');  PostSaveFcn=alt_dspbuilder_block_saved(gcb);  NameChangeFcn=alt_dspbuilder_block_renamed(gcb);
      mask Help: helpview(char(com.altera.dspbuilder.simulation.Cache.getBlockTemplate('BlockFactory', 'com.altera.dspbuilder.blockset.arithmetic.SquareRoot').getHelpFile))
      mask StyleString: popup(Signed Integer|Unsigned Integer|Signed Fractional|Unsigned Fractional),edit,edit,edit,edit,checkbox,checkbox,checkbox
      mask CallbackString: |||||alt_dspbuilder_update_gui('BlockFactory', 'com.altera.dspbuilder.blockset.arithmetic.SquareRoot', 'use_remain', 5);||
      mask TabNameString: Main,Main,Main,Main,Main,Optional Ports,Optional Ports,Optional Ports
      mask Display:
      | port_label('input', 1, 'd(7:0)');
      | port_label('output', 1, 'q(3:0)');
      | plot([0.1875 0.375 0.4375 0.5 1], [0.375 0.375 0.0625 1 1])
  State Machine : S-Function  LoadFcn=alt_dspbuilder_load_block(gcb, 'BlockFactory', 'com.altera.dspbuilder.blockset.statemachinefunctions.StateMachine');  FunctionName=sGeneric  Parameters=Inputs States db_entity VHDL_ARCHITECTURE reset_state all_states all_inputs all_conditions input_names output_names is_initialized pipeline_display  EnableBusSupport=off  mask(State Machine AlteraBlockset){Inputs=6, States=6, db_entity=, VHDL_ARCHITECTURE=uninitialized, reset_state=, all_states=, all_inputs=, all_conditions=, input_names=reset in2 in3 in4 in5 in6, output_names=out1 out2 out3 out4 out5 out6, is_initialized=off, pipeline_display=1}
      mask prompts: pipeline_display "Number Of Pipeline Stages (Calculated)"
      mask help:
      | Represents a one-hot Moore style state machine where the output is equal to the current state.
      |
      | N.B. This block is deprecated. The State Machine Editor block should be used in new designs in preference to this block.
      mask init:
      | alt_dspbuilder_state_machine_init_callback('BlockFactory', 'com.altera.dspbuilder.blockset.statemachinefunctions.StateMachine', { Inputs States db_entity VHDL_ARCHITECTURE reset_state all_states all_inputs all_conditions input_names output_names is_initialized pipeline_display });
      settings: CopyFcn=alt_dspbuilder_add_block(gcb, 'BlockFactory', 'com.altera.dspbuilder.blockset.statemachinefunctions.StateMachine');  DeleteFcn=com.altera.dspbuilder.simulation.Mask.delete(gcb);  UndoDeleteFcn=alt_dspbuilder_add_block(gcb, 'BlockFactory', 'com.altera.dspbuilder.blockset.statemachinefunctions.StateMachine');  PostSaveFcn=alt_dspbuilder_block_saved(gcb);  NameChangeFcn=alt_dspbuilder_block_renamed(gcb);
      settings: OpenFcn=|
      | com.altera.dspbuilder.simulation.Mask.simpleInit('BlockFactory', 'com.altera.dspbuilder.blockset.statemachinefunctions.StateMachine', bdroot(gcb), gcb);
      | alt_dspbuilder_state_machine_run(gcb)
      mask Help: helpview(char(com.altera.dspbuilder.simulation.Cache.getBlockTemplate('BlockFactory', 'com.altera.dspbuilder.blockset.statemachinefunctions.StateMachine').getHelpFile))
      mask Display:
      | port_label('input', 1, 'reset');
      | port_label('input', 2, 'in2');
      | port_label('input', 3, 'in3');
      | port_label('input', 4, 'in4');
      | port_label('input', 5, 'in5');
      | port_label('input', 6, 'in6');
      | port_label('output', 1, 'out1');
      | port_label('output', 2, 'out2');
      | port_label('output', 3, 'out3');
      | port_label('output', 4, 'out4');
      | port_label('output', 5, 'out5');
      | port_label('output', 6, 'out6');
      | disp('');
  State Machine Editor : S-Function  LoadFcn=alt_dspbuilder_load_block(gcb, 'BlockFactory', 'com.altera.dspbuilder.blockset.statemachinefunctions.StateMachineEditor');  InitFcn=alt_dspbuilder_internal_init_blackbox_flow;  FunctionName=sGeneric  Parameters=entityName smf_file use_dynamic_feedthrough_data inNames inBwls inBwrs inTypes inDelayed outNames outBwls outBwrs outTypes n_input_port n_output_port array_clocks resetNames resetTypes resetLengths xmlmapfile vofile use_systemC_model is_megacore smf_variation  EnableBusSupport=off  mask(Integrated Quartus State Machine AlteraBlockset){entityName=, smf_file=, use_dynamic_feedthrough_data=on, inNames=, inBwls=, inBwrs=, inTypes=, inDelayed=, outNames=, outBwls=, outBwrs=, outTypes=, n_input_port=0, n_output_port=0, array_clocks=, resetNames=, resetTypes=, resetLengths=, xmlmapfile=SimgenCMap.xml, vofile=test_core.vo, use_systemC_model=off, is_megacore=off, smf_variation=}
      mask prompts: entityName "Entity Name"; inNames "Input port names"; inBwls "Input Bitwidth lefts"; inBwrs "Input Bitwidth rights"; inTypes "Input Types"; inDelayed "Input Delayed Flags"; outNames "Output port names"; outBwls "Output Bitwidth lefts"; outBwrs "Output Bitwidth rights"; outTypes "Output Types"; resetNames "array_clocks"; resetTypes "array_clocks"; resetLengths "array_clocks"; use_systemC_model "Use SystemC bit-accurate model"
      mask help: Provides access to the Quartus II State Machine Editor which allows you to create graphic representations of state machines for use in your design.
      mask init:
      | alt_dspbuilder_init('BlockFactory', 'com.altera.dspbuilder.blockset.statemachinefunctions.StateMachineEditor', { entityName smf_file use_dynamic_feedthrough_data inNames inBwls inBwrs inTypes inDelayed outNames outBwls outBwrs outTypes n_input_port n_output_port array_clocks resetNames resetTypes resetLengths xmlmapfile vofile use_systemC_model is_megacore smf_variation });
      settings: CopyFcn=alt_dspbuilder_add_block(gcb, 'BlockFactory', 'com.altera.dspbuilder.blockset.statemachinefunctions.StateMachineEditor');  DeleteFcn=com.altera.dspbuilder.simulation.Mask.delete(gcb);  UndoDeleteFcn=alt_dspbuilder_add_block(gcb, 'BlockFactory', 'com.altera.dspbuilder.blockset.statemachinefunctions.StateMachineEditor');  PostSaveFcn=alt_dspbuilder_block_saved(gcb);  NameChangeFcn=alt_dspbuilder_block_renamed(gcb);
      settings: OpenFcn=|
      | com.altera.dspbuilder.simulation.Mask.simpleInit('BlockFactory', 'com.altera.dspbuilder.blockset.statemachinefunctions.StateMachineEditor', bdroot(gcb), gcb);
      | alt_dspbuilder_launch_state_machine_editor(gcb, 0)
      mask Help: helpview(char(com.altera.dspbuilder.simulation.Cache.getBlockTemplate('BlockFactory', 'com.altera.dspbuilder.blockset.statemachinefunctions.StateMachineEditor').getHelpFile))
      mask Display: disp('Graphical State Machine Editor');
  Subsystem Builder : S-Function  LoadFcn=alt_dspbuilder_load_block(gcb, 'BlockFactory', 'com.altera.dspbuilder.blockset.altlab.SubSystemBuilder');  InitFcn=alt_dspbuilder_internal_init_altlab_flow;  FunctionName=sNoOp  Parameters=entityName inNames inBwls inBwrs inTypes inDelayed outNames outBwls outBwrs outTypes resetNames resetTypes resetLengths  EnableBusSupport=off  mask(Subsystem Builder AlteraBlockset){entityName=, inNames=, inBwls=, inBwrs=, inTypes=, inDelayed=, outNames=, outBwls=, outBwrs=, outTypes=, resetNames=, resetTypes=, resetLengths=}
      mask prompts: entityName "Entity Name"; inNames "Input port names"; inBwls "Input Bitwidth lefts"; inBwrs "Input Bitwidth rights"; inTypes "Input Types"; inDelayed "Input Delayed Flags"; outNames "Output port names"; outBwls "Output Bitwidth lefts"; outBwrs "Output Bitwidth rights"; outTypes "Output Types"; resetNames "array_clocks"; resetTypes "array_clocks"; resetLengths "array_clocks"
      mask help: Allows you to build black box subsystems that synthesize using user-supplied VHDL and simulate using non-DSP Builder Simulink blocks. This is an alternative to using HDL Import and can give better simulation speed. You can also use this block if HDL Import cannot be used due to unsupported megafunctions or LPMs.
      mask init:
      | alt_dspbuilder_init('BlockFactory', 'com.altera.dspbuilder.blockset.altlab.SubSystemBuilder', { entityName inNames inBwls inBwrs inTypes inDelayed outNames outBwls outBwrs outTypes resetNames resetTypes resetLengths });
      settings: CopyFcn=alt_dspbuilder_add_block(gcb, 'BlockFactory', 'com.altera.dspbuilder.blockset.altlab.SubSystemBuilder');  DeleteFcn=com.altera.dspbuilder.simulation.Mask.delete(gcb);  UndoDeleteFcn=alt_dspbuilder_add_block(gcb, 'BlockFactory', 'com.altera.dspbuilder.blockset.altlab.SubSystemBuilder');  PostSaveFcn=alt_dspbuilder_block_saved(gcb);  NameChangeFcn=alt_dspbuilder_block_renamed(gcb);
      settings: OpenFcn=|
      | com.altera.dspbuilder.simulation.Mask.simpleInit('BlockFactory', 'com.altera.dspbuilder.blockset.altlab.SubSystemBuilder', bdroot(gcb), gcb);
      | alt_dspbuilder_build_subsystem('alt_dspbuilder_build_subsystem')
      mask Help: helpview(char(com.altera.dspbuilder.simulation.Cache.getBlockTemplate('BlockFactory', 'com.altera.dspbuilder.blockset.altlab.SubSystemBuilder').getHelpFile))
      mask Display: image(imread('SUBSYSBUILD.bmp', 'bmp'));
  Sum of Products : S-Function  LoadFcn=alt_dspbuilder_load_block(gcb, 'BlockFactory', 'com.altera.dspbuilder.blockset.arithmetic.SumOfProducts');  FunctionName=sGeneric  Parameters=BusType InputBwl InputBwr number_of_coefficients CoefBwl CoefBwr coefficients pipeline pipeline_display full_resolution OutputBwl OutputBwr TruncateLsb implementation use_ena use_aclr  EnableBusSupport=off  mask(SumOfProducts AlteraBlockset){BusType=Signed Integer, InputBwl=8, InputBwr=0, number_of_coefficients=4, CoefBwl=8, CoefBwr=0, coefficients=[1 2 3 4 5 6 7 8], pipeline=0, pipeline_display=0, full_resolution=on, OutputBwl=8, OutputBwr=0, TruncateLsb=0, implementation=Auto, use_ena=off, use_aclr=off}
      mask prompts: BusType "Bus Type"; InputBwl "Input Data Number of Bits"; number_of_coefficients "Number of Coefficients (1-8)"; CoefBwl "Coefficient Number of Bits"; CoefBwr "[].[Number Of Bits]"; coefficients "Signed Integer Fixed-Coefficient Values (C_i)"; pipeline "Number of Pipeline Stages"; pipeline_display "Number Of Pipeline Stages (Calculated)"; full_resolution "Full Resolution for Output Result"; OutputBwl "Output Number of Bits"; TruncateLsb "Output Truncated LSB"; implementation "FPGA Implementation"; use_ena "Use Enable Port (ena)"; use_aclr "Use Asynchronous Clear Port (aclr)"
      mask help:
      | Implements the following expression:
      |
      |  q = a(0)C0 + ... + a(i)Ci + ... + a(n-1)Cn-1
      |
      |  a(i) : Signed integer input data
      |  Ci   : Constant signed integer coefficients
      |  n    : Number of coefficients (1-8)
      |
      | Disable "Full Resolution for Output Result" to truncate output. Output Number of Bits then specifies the width of the output, and Output Truncated LSB the number of least-significant bits to be dropped.
      mask init:
      | alt_dspbuilder_init('BlockFactory', 'com.altera.dspbuilder.blockset.arithmetic.SumOfProducts', { BusType InputBwl InputBwr number_of_coefficients CoefBwl CoefBwr coefficients pipeline pipeline_display get_param(gcb, 'full_resolution') OutputBwl OutputBwr TruncateLsb implementation use_ena use_aclr });
      settings: CopyFcn=alt_dspbuilder_add_block(gcb, 'BlockFactory', 'com.altera.dspbuilder.blockset.arithmetic.SumOfProducts');  DeleteFcn=com.altera.dspbuilder.simulation.Mask.delete(gcb);  UndoDeleteFcn=alt_dspbuilder_add_block(gcb, 'BlockFactory', 'com.altera.dspbuilder.blockset.arithmetic.SumOfProducts');  PostSaveFcn=alt_dspbuilder_block_saved(gcb);  NameChangeFcn=alt_dspbuilder_block_renamed(gcb);
